simulink model "Test1_3"  (R2021a)
(part 1 of 2)
settings: Solver=FixedStepAuto  StartTime=0  StopTime=0.2  FixedStep=0.2  RelTol=1e-3
libraries: spsDistributedParametersLineLib x74, spsThreePhaseSeriesRLCLoadLib x25, spsThreePhaseVIMeasurementLib x5, spsGroundLib x1, spsThreePhaseSourceLib x1, spsSeriesRLCBranchLib x1, spspowerguiLib x1
settings Model: Creator=Admin  LastModifiedBy=Admin

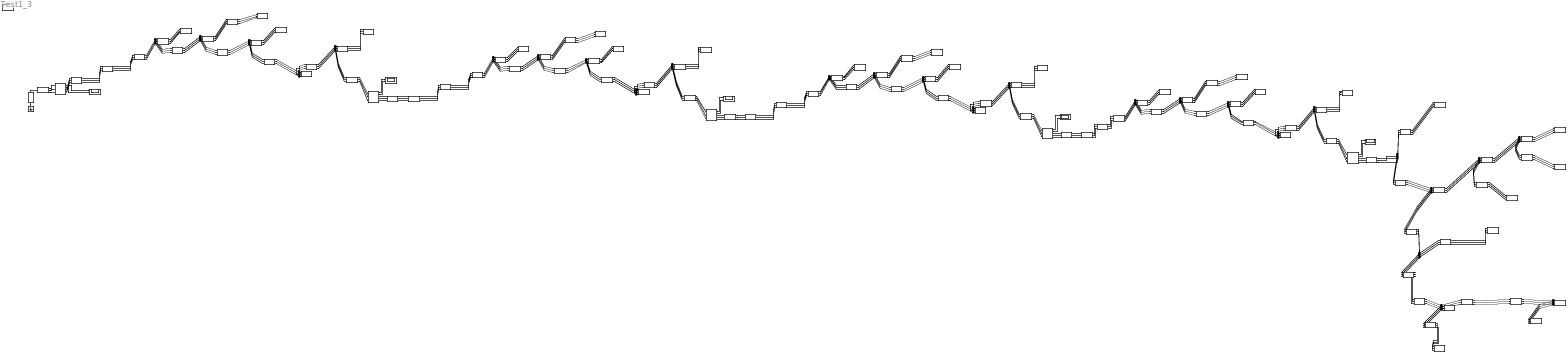
== system Test1_3 ==
  Ground : spsGroundLib/Ground  LConnTagsString=a
  Line 1 : spsDistributedParametersLineLib/Distributed Parameters Line  Phases=3  Length=0.24  Frequency=50  Resistance=[0.646656091154803 0.0486237908083191 0.0486712220507153;0.0486237908083191 0.646561225344642 0.0486237934466192;0.0486712220507153 0.0486237934466192 0.646656091154803]  Inductance=[0.00282448912315926 0.00133270803418135 0.00132951476746136;0.00133270803418135 0.00282479813276775 0.00133799988507366;0.00132951476746136 0.00133799988507366 0.00282448912315926]  Capacitance=[7.89543174552926e-09 -1.85986777702161e-09 -1.7901190036642e-09;-1.85986777702161e-09 7.82540023894543e-09 -1.8957321828871e-09;-1.7901190036642e-09 -1.8957321828871e-09 7.91264394645417e-09]  x1=[222.015092797367 9898.99389241635 9898.51429142449;314.159265358979 314.159265358979 314.159265358979;-3.07254403430719 -0.183299396266418 -1.75413682242909]  x2=[222.020723483214 9898.49942617451 9898.02069734636;314.159265358979 314.159265358979 314.159265358979;-3.07254410726608 -0.183335294452607 -1.75417253731169]  x3=[0.199348875998997 21.8526585587068 22.0454388073924;314.159265358979 314.159265358979 314.159265358979;-3.13045863300509 -0.176900643269076 -1.74803218325065]  x4=[0.189523343990307 28.5168236303326 28.7082767154191;314.159265358979 314.159265358979 314.159265358979;-3.01199407510197 -0.188487989154 -1.75911017054267]  x5=1.14995345102668e-06  V1=ones(3,3)  V2=ones(3,3)  I1=ones(3,3)  I2=ones(3,3)  nHarmo=1  Measurements=None  Decoupling=off  VsMag0=0  VrMag0=0  VsAngle0=0  VrAngle0=0  IsMag0=0  IrMag0=0  IsAngle0=0  IrAngle0=0
      settings: SourceProductBaseCode=PS
  Line 10 : spsDistributedParametersLineLib/Distributed Parameters Line  Phases=3  Length=0.17001  Frequency=50  Resistance=[0.646656091154803 0.0486237908083191 0.0486712220507153;0.0486237908083191 0.646561225344642 0.0486237934466192;0.0486712220507153 0.0486237934466192 0.646656091154803]  Inductance=[0.00282448912315926 0.00133270803418135 0.00132951476746136;0.00133270803418135 0.00282479813276775 0.00133799988507366;0.00132951476746136 0.00133799988507366 0.00282448912315926]  Capacitance=[7.89543174552926e-09 -1.85986777702161e-09 -1.7901190036642e-09;-1.85986777702161e-09 7.82540023894543e-09 -1.8957321828871e-09;-1.7901190036642e-09 -1.8957321828871e-09 7.91264394645417e-09]  x1=[221.972317308412 9904.72208898904 9904.23123830907;314.159265358979 314.159265358979 314.159265358979;-3.07236720751226 -0.182923549459791 -1.75376288206444]  x2=[221.972231728308 9904.60473873258 9904.1140740022;314.159265358979 314.159265358979 314.159265358979;-3.07237120414623 -0.182927320155413 -1.75376660852685]  x3=[0.191402295206027 24.3117265787812 24.5037810965484;314.159265358979 314.159265358979 314.159265358979;-3.07696679484423 -0.169300487327628 -1.74025339126651]  x4=[0.196725593404522 26.095480950671 26.2879206642852;314.159265358979 314.159265358979 314.159265358979;-3.06814848425652 -0.195815367857081 -1.76655565060886]  x5=8.14598275871021e-07  V1=ones(3,3)  V2=ones(3,3)  I1=ones(3,3)  I2=ones(3,3)  nHarmo=1  Measurements=None  Decoupling=off  VsMag0=0  VrMag0=0  VsAngle0=0  VrAngle0=0  IsMag0=0  IrMag0=0  IsAngle0=0  IrAngle0=0
      settings: SourceProductBaseCode=PS
  Line 11 : spsDistributedParametersLineLib/Distributed Parameters Line  Phases=3  Length=0.27998  Frequency=50  Resistance=[0.646656091154803 0.0486237908083191 0.0486712220507153;0.0486237908083191 0.646561225344642 0.0486237934466192;0.0486712220507153 0.0486237934466192 0.646656091154803]  Inductance=[0.00282448912315926 0.00133270803418135 0.00132951476746136;0.00133270803418135 0.00282479813276775 0.00133799988507366;0.00132951476746136 0.00133799988507366 0.00282448912315926]  Capacitance=[7.89543174552926e-09 -1.85986777702161e-09 -1.7901190036642e-09;-1.85986777702161e-09 7.82540023894543e-09 -1.8957321828871e-09;-1.7901190036642e-09 -1.8957321828871e-09 7.91264394645417e-09]  x1=[221.964400678937 9906.160798162 9905.66713429306;314.159265358979 314.159265358979 314.159265358979;-3.07250282075598 -0.182996515026566 -1.75383646753957]  x2=[221.972317308412 9904.72208898904 9904.23123830907;314.159265358979 314.159265358979 314.159265358979;-3.07253274376391 -0.183055057139632 -1.75389451493028]  x3=[0.189343973964793 18.3203804193673 18.510412001508;314.159265358979 314.159265358979 314.159265358979;3.11070886720037 -0.071966798330211 -1.64431562110163]  x4=[0.200581894562315 32.2574047158268 32.4491284475579;314.159265358979 314.159265358979 314.159265358979;-2.97858619624838 -0.246275175394318 -1.8165359331067]  x5=1.34151653007687e-06  V1=ones(3,3)  V2=ones(3,3)  I1=ones(3,3)  I2=ones(3,3)  nHarmo=1  Measurements=None  Decoupling=off  VsMag0=0  VrMag0=0  VsAngle0=0  VrAngle0=0  IsMag0=0  IrMag0=0  IsAngle0=0  IrAngle0=0
      settings: SourceProductBaseCode=PS
  Line 12 : spsDistributedParametersLineLib/Distributed Parameters Line  Phases=3  Length=0.01  Frequency=50  Resistance=[0.646656091154803 0.0486237908083191 0.0486712220507153;0.0486237908083191 0.646561225344642 0.0486237934466192;0.0486712220507153 0.0486237934466192 0.646656091154803]  Inductance=[0.00282448912315926 0.00133270803418135 0.00132951476746136;0.00133270803418135 0.00282479813276775 0.00133799988507366;0.00132951476746136 0.00133799988507366 0.00282448912315926]  Capacitance=[7.89543174552926e-09 -1.85986777702161e-09 -1.7901190036642e-09;-1.85986777702161e-09 7.82540023894543e-09 -1.8957321828871e-09;-1.7901190036642e-09 -1.8957321828871e-09 7.91264394645417e-09]  x1=[221.964117196425 9906.21216439256 9905.71839999673;314.159265358979 314.159265358979 314.159265358979;-3.0720953535524 -0.182671566045166 -1.75351122886673]  x2=[221.964400678937 9906.160798162 9905.66713429306;314.159265358979 314.159265358979 314.159265358979;-3.0720964237639 -0.182673659307702 -1.75351330448492]  x3=[0.189369051494013 18.3268185948226 18.5169580964303;314.159265358979 314.159265358979 314.159265358979;3.11110535727251 -0.0716738702183169 -1.64402223817255]  x4=[0.200609281456702 32.2696425742855 32.4615173065927;314.159265358979 314.159265358979 314.159265358979;-2.97774579617266 -0.245633417397122 -1.81589354797315]  x5=4.79147271261115e-08  V1=ones(3,3)  V2=ones(3,3)  I1=ones(3,3)  I2=ones(3,3)  nHarmo=1  Measurements=None  Decoupling=off  VsMag0=0  VrMag0=0  VsAngle0=0  VrAngle0=0  IsMag0=0  IrMag0=0  IsAngle0=0  IrAngle0=0
      settings: SourceProductBaseCode=PS
  Line 13 : spsDistributedParametersLineLib/Distributed Parameters Line  Phases=3  Length=0.04  Frequency=50  Resistance=[0.646656091154803 0.0486237908083191 0.0486712220507153;0.0486237908083191 0.646561225344642 0.0486237934466192;0.0486712220507153 0.0486237934466192 0.646656091154803]  Inductance=[0.00282448912315926 0.00133270803418135 0.00132951476746136;0.00133270803418135 0.00282479813276775 0.00133799988507366;0.00132951476746136 0.00133799988507366 0.00282448912315926]  Capacitance=[7.89543174552926e-09 -1.85986777702161e-09 -1.7901190036642e-09;-1.85986777702161e-09 7.82540023894543e-09 -1.8957321828871e-09;-1.7901190036642e-09 -1.8957321828871e-09 7.91264394645417e-09]  x1=[221.962982765951 9906.41761558248 9905.92344904545;314.159265358979 314.159265358979 314.159265358979;-3.07213623026815 -0.182699066907734 -1.75353883444]  x2=[221.964117196425 9906.21216439257 9905.71839999674;314.159265358979 314.159265358979 314.159265358979;-3.07214051211882 -0.182707441560263 -1.75354713853278]  x3=[0.189366364091302 18.3265238939544 18.5166548882844;314.159265358979 314.159265358979 314.159265358979;3.11100214349639 -0.071765112869428 -1.64411349403723]  x4=[0.200606435854495 32.2687271891192 32.4605884092911;314.159265358979 314.159265358979 314.159265358979;-2.97777486414768 -0.245658643022115 -1.81591879618078]  x5=1.91658908504446e-07  V1=ones(3,3)  V2=ones(3,3)  I1=ones(3,3)  I2=ones(3,3)  nHarmo=1  Measurements=None  Decoupling=off  VsMag0=0  VrMag0=0  VsAngle0=0  VrAngle0=0  IsMag0=0  IrMag0=0  IsAngle0=0  IrAngle0=0
      settings: SourceProductBaseCode=PS
  Line 14 : spsDistributedParametersLineLib/Distributed Parameters Line  Phases=3  Length=0.24  Frequency=50  Resistance=[0.646656091154803 0.0486237908083191 0.0486712220507153;0.0486237908083191 0.646561225344642 0.0486237934466192;0.0486712220507153 0.0486237934466192 0.646656091154803]  Inductance=[0.00282448912315926 0.00133270803418135 0.00132951476746136;0.00133270803418135 0.00282479813276775 0.00133799988507366;0.00132951476746136 0.00133799988507366 0.00282448912315926]  Capacitance=[7.89543174552926e-09 -1.85986777702161e-09 -1.7901190036642e-09;-1.85986777702161e-09 7.82540023894543e-09 -1.8957321828871e-09;-1.7901190036642e-09 -1.8957321828871e-09 7.91264394645417e-09]  x1=[221.973522275872 9925.87360304901 9925.32102641094;314.159265358979 314.159265358979 314.159265358979;-3.0717657082313 -0.182168328973665 -1.75301176636206]  x2=[221.977087028903 9923.47138515495 9922.92903593915;314.159265358979 314.159265358979 314.159265358979;-3.07183596694289 -0.182262149538667 -1.7531047608717]  x3=[0.166701605313396 12.4551511660944 12.6489512436628;314.159265358979 314.159265358979 314.159265358979;3.08491891689076 0.154861392301933 -1.42392082854132]  x4=[0.223729457265582 38.9654485817741 39.1305023133519;314.159265358979 314.159265358979 314.159265358979;-2.97799775422241 -0.288316615314577 -1.8579203605478]  x5=1.14995345102668e-06  V1=ones(3,3)  V2=ones(3,3)  I1=ones(3,3)  I2=ones(3,3)  nHarmo=1  Measurements=None  Decoupling=off  VsMag0=0  VrMag0=0  VsAngle0=0  VrAngle0=0  IsMag0=0  IrMag0=0  IsAngle0=0  IrAngle0=0
      settings: SourceProductBaseCode=PS
  Line 15 : spsDistributedParametersLineLib/Distributed Parameters Line  Phases=3  Length=0.17  Frequency=50  Resistance=[0.646656091154803 0.0486237908083191 0.0486712220507153;0.0486237908083191 0.646561225344642 0.0486237934466192;0.0486712220507153 0.0486237934466192 0.646656091154803]  Inductance=[0.00282448912315926 0.00133270803418135 0.00132951476746136;0.00133270803418135 0.00282479813276775 0.00133799988507366;0.00132951476746136 0.00133799988507366 0.00282448912315926]  Capacitance=[7.89543174552926e-09 -1.85986777702161e-09 -1.7901190036642e-09;-1.85986777702161e-09 7.82540023894543e-09 -1.8957321828871e-09;-1.7901190036642e-09 -1.8957321828871e-09 7.91264394645417e-09]  x1=[221.944814686174 9946.32776513441 9945.69460604376;314.159265358979 314.159265358979 314.159265358979;-3.07104566344104 -0.181319930646415 -1.75217030363738]  x2=[221.944466798057 9946.09949773542 9945.46678149026;314.159265358979 314.159265358979 314.159265358979;-3.07105307589 -0.181324540973944 -1.75217483471912]  x3=[0.188869541515534 23.713943126835 23.9061742104411;314.159265358979 314.159265358979 314.159265358979;-3.07669220860616 -0.147173041953311 -1.71830841602994]  x4=[0.199211853754603 26.9264377171524 27.1194193511748;314.159265358979 314.159265358979 314.159265358979;-3.0659487506894 -0.211587070451044 -1.78221448870695]  x5=8.14550361143895e-07  V1=ones(3,3)  V2=ones(3,3)  I1=ones(3,3)  I2=ones(3,3)  nHarmo=1  Measurements=None  Decoupling=off  VsMag0=0  VrMag0=0  VsAngle0=0  VrAngle0=0  IsMag0=0  IrMag0=0  IsAngle0=0  IrAngle0=0
      settings: SourceProductBaseCode=PS
  Line 16 : spsDistributedParametersLineLib/Distributed Parameters Line  Phases=3  Length=0.27998  Frequency=50  Resistance=[0.646656091154803 0.0486237908083191 0.0486712220507153;0.0486237908083191 0.646561225344642 0.0486237934466192;0.0486712220507153 0.0486237934466192 0.646656091154803]  Inductance=[0.00282448912315926 0.00133270803418135 0.00132951476746136;0.00133270803418135 0.00282479813276775 0.00133799988507366;0.00132951476746136 0.00133799988507366 0.00282448912315926]  Capacitance=[7.89543174552926e-09 -1.85986777702161e-09 -1.7901190036642e-09;-1.85986777702161e-09 7.82540023894543e-09 -1.8957321828871e-09;-1.7901190036642e-09 -1.8957321828871e-09 7.91264394645417e-09]  x1=[221.939122386853 9950.29824850916 9949.65104582546;314.159265358979 314.159265358979 314.159265358979;-3.07108819087539 -0.181309560588363 -1.75216142668549]  x2=[221.944814686174 9946.32776513441 9945.69460604376;314.159265358979 314.159265358979 314.159265358979;-3.07121121474554 -0.181451450284761 -1.7523019484731]  x3=[0.153632894301808 9.09985631328812 9.23355063958161;314.159265358979 314.159265358979 314.159265358979;3.01164471861859 0.584493625789448 -1.00502772438115]  x4=[0.239442202240828 44.5100191865775 44.6743802062215;314.159265358979 314.159265358979 314.159265358979;-2.94342659054599 -0.323766194698098 -1.89335245445794]  x5=1.34151653007687e-06  V1=ones(3,3)  V2=ones(3,3)  I1=ones(3,3)  I2=ones(3,3)  nHarmo=1  Measurements=None  Decoupling=off  VsMag0=0  VrMag0=0  VsAngle0=0  VrAngle0=0  IsMag0=0  IrMag0=0  IsAngle0=0  IrAngle0=0
      settings: SourceProductBaseCode=PS
  Line 17 : spsDistributedParametersLineLib/Distributed Parameters Line  Phases=3  Length=0.01  Frequency=50  Resistance=[0.646656091154803 0.0486237908083191 0.0486712220507153;0.0486237908083191 0.646561225344642 0.0486237934466192;0.0486712220507153 0.0486237934466192 0.646656091154803]  Inductance=[0.00282448912315926 0.00133270803418135 0.00132951476746136;0.00133270803418135 0.00282479813276775 0.00133799988507366;0.00132951476746136 0.00133799988507366 0.00282448912315926]  Capacitance=[7.89543174552926e-09 -1.85986777702161e-09 -1.7901190036642e-09;-1.85986777702161e-09 7.82540023894543e-09 -1.8957321828871e-09;-1.7901190036642e-09 -1.8957321828871e-09 7.91264394645417e-09]  x1=[221.938918408942 9950.44004469309 9949.79234030743;314.159265358979 314.159265358979 314.159265358979;-3.07067739832622 -0.180981636475063 -1.75183324404407]  x2=[221.939122386853 9950.29824850916 9949.65104582545;314.159265358979 314.159265358979 314.159265358979;-3.07068179388331 -0.1809867048695 -1.75183826363084]  x3=[0.153654926726157 9.10373918144453 9.23754358970651;314.159265358979 314.159265358979 314.159265358979;3.01204871867404 0.584577230830885 -1.00493947494426]  x4=[0.239480161563136 44.5300262788079 44.6945783680464;314.159265358979 314.159265358979 314.159265358979;-2.94258448112311 -0.323134577726176 -1.89272027652599]  x5=4.79147271261115e-08  V1=ones(3,3)  V2=ones(3,3)  I1=ones(3,3)  I2=ones(3,3)  nHarmo=1  Measurements=None  Decoupling=off  VsMag0=0  VrMag0=0  VsAngle0=0  VrAngle0=0  IsMag0=0  IrMag0=0  IsAngle0=0  IrAngle0=0
      settings: SourceProductBaseCode=PS
  Line 18 : spsDistributedParametersLineLib/Distributed Parameters Line  Phases=3  Length=0.04  Frequency=50  Resistance=[0.646656091154803 0.0486237908083191 0.0486712220507153;0.0486237908083191 0.646561225344642 0.0486237934466192;0.0486712220507153 0.0486237934466192 0.646656091154803]  Inductance=[0.00282448912315926 0.00133270803418135 0.00132951476746136;0.00133270803418135 0.00282479813276775 0.00133799988507366;0.00132951476746136 0.00133799988507366 0.00282448912315926]  Capacitance=[7.89543174552926e-09 -1.85986777702161e-09 -1.7901190036642e-09;-1.85986777702161e-09 7.82540023894543e-09 -1.8957321828871e-09;-1.7901190036642e-09 -1.8957321828871e-09 7.91264394645417e-09]  x1=[221.938102037263 9951.00721775521 9950.35750648626;314.159265358979 314.159265358979 314.159265358979;-3.07070497360592 -0.180997238037415 -1.75184907495375]  x2=[221.938918408942 9950.44004469309 9949.79234030743;314.159265358979 314.159265358979 314.159265358979;-3.07072255689264 -0.18101751199016 -1.75186915371012]  x3=[0.153653451843419 9.10388021603596 9.23769760590279;314.159265358979 314.159265358979 314.159265358979;3.01194864834173 0.584398219446076 -1.00511674278829]  x4=[0.239477198969098 44.5290201004338 44.6935581340705;314.159265358979 314.159265358979 314.159265358979;-2.9426134072445 -0.323160639687177 -1.89274636652624]  x5=1.91658908504446e-07  V1=ones(3,3)  V2=ones(3,3)  I1=ones(3,3)  I2=ones(3,3)  nHarmo=1  Measurements=None  Decoupling=off  VsMag0=0  VrMag0=0  VsAngle0=0  VrAngle0=0  IsMag0=0  IrMag0=0  IsAngle0=0  IrAngle0=0
      settings: SourceProductBaseCode=PS
  Line 19 : spsDistributedParametersLineLib/Distributed Parameters Line  Phases=3  Length=0.02  Frequency=50  Resistance=[0.646656091154803 0.0486237908083191 0.0486712220507153;0.0486237908083191 0.646561225344642 0.0486237934466192;0.0486712220507153 0.0486237934466192 0.646656091154803]  Inductance=[0.00282448912315926 0.00133270803418135 0.00132951476746136;0.00133270803418135 0.00282479813276775 0.00133799988507366;0.00132951476746136 0.00133799988507366 0.00282448912315926]  Capacitance=[7.89543174552926e-09 -1.85986777702161e-09 -1.7901190036642e-09;-1.85986777702161e-09 7.82540023894543e-09 -1.8957321828871e-09;-1.7901190036642e-09 -1.8957321828871e-09 7.91264394645417e-09]  x1=[221.973522275872 9925.87360304901 9925.32102641094;314.159265358979 314.159265358979 314.159265358979;-3.07143454541088 -0.181905241862953 -1.75274842881105]  x2=[221.973516698645 9925.86853585086 9925.31596800554;314.159265358979 314.159265358979 314.159265358979;-3.07143471408227 -0.181905377807733 -1.75274856290877]  x3=[0.193101763304672 24.9432757831222 25.1357901814941;314.159265358979 314.159265358979 314.159265358979;-3.07278996594042 -0.176459776755126 -1.74734653840281]  x4=[0.195053219699961 25.5768094426152 25.7694636724105;314.159265358979 314.159265358979 314.159265358979;-3.07012280847577 -0.187239577579629 -1.75804126304697]  x5=9.5829454252223e-08  V1=ones(3,3)  V2=ones(3,3)  I1=ones(3,3)  I2=ones(3,3)  nHarmo=1  Measurements=None  Decoupling=off  VsMag0=0  VrMag0=0  VsAngle0=0  VrAngle0=0  IsMag0=0  IrMag0=0  IsAngle0=0  IrAngle0=0
      settings: SourceProductBaseCode=PS
  Line 2 : spsDistributedParametersLineLib/Distributed Parameters Line  Phases=3  Length=0.02  Frequency=50  Resistance=[0.646656091154803 0.0486237908083191 0.0486712220507153;0.0486237908083191 0.646561225344642 0.0486237934466192;0.0486712220507153 0.0486237934466192 0.646656091154803]  Inductance=[0.00282448912315926 0.00133270803418135 0.00132951476746136;0.00133270803418135 0.00282479813276775 0.00133799988507366;0.00132951476746136 0.00133799988507366 0.00282448912315926]  Capacitance=[7.89543174552926e-09 -1.85986777702161e-09 -1.7901190036642e-09;-1.85986777702161e-09 7.82540023894543e-09 -1.8957321828871e-09;-1.7901190036642e-09 -1.8957321828871e-09 7.91264394645417e-09]  x1=[222.015092797367 9898.99389241635 9898.51429142449;314.159265358979 314.159265358979 314.159265358979;-3.07221287148677 -0.183036309155706 -1.75387348487807]  x2=[222.015083980034 9898.98951139534 9898.50991976959;314.159265358979 314.159265358979 314.159265358979;-3.07221300948614 -0.183036365995476 -1.75387354026733]  x3=[0.193270328840676 24.9423814090567 25.1345622020492;314.159265358979 314.159265358979 314.159265358979;-3.0727848843541 -0.177077853265056 -1.74796182768062]  x4=[0.194957058349762 25.4410435312021 25.6333539339617;314.159265358979 314.159265358979 314.159265358979;-3.07167592078859 -0.188901712894827 -1.75969386949824]  x5=9.5829454252223e-08  V1=ones(3,3)  V2=ones(3,3)  I1=ones(3,3)  I2=ones(3,3)  nHarmo=1  Measurements=None  Decoupling=off  VsMag0=0  VrMag0=0  VsAngle0=0  VrAngle0=0  IsMag0=0  IrMag0=0  IsAngle0=0  IrAngle0=0
      settings: SourceProductBaseCode=PS
  Line 20 : spsDistributedParametersLineLib/Distributed Parameters Line  Phases=3  Length=0.5  Frequency=50  Resistance=[0.646656091154803 0.0486237908083191 0.0486712220507153;0.0486237908083191 0.646561225344642 0.0486237934466192;0.0486712220507153 0.0486237934466192 0.646656091154803]  Inductance=[0.00282448912315926 0.00133270803418135 0.00132951476746136;0.00133270803418135 0.00282479813276775 0.00133799988507366;0.00132951476746136 0.00133799988507366 0.00282448912315926]  Capacitance=[7.89543174552926e-09 -1.85986777702161e-09 -1.7901190036642e-09;-1.85986777702161e-09 7.82540023894543e-09 -1.8957321828871e-09;-1.7901190036642e-09 -1.8957321828871e-09 7.91264394645417e-09]  x1=[221.966143238206 9931.00249399023 9930.42838033784;314.159265358979 314.159265358979 314.159265358979;-3.07200630035913 -0.18228019640756 -1.75312569202443]  x2=[221.973522275872 9925.87360304901 9925.32102641094;314.159265358979 314.159265358979 314.159265358979;-3.07215708247362 -0.182479250104506 -1.7533229834678]  x3=[0.165753744342144 12.2073465655838 12.3991659443851;314.159265358979 314.159265358979 314.159265358979;3.08150867253815 0.172561744291717 -1.40667076257851]  x4=[0.224703111158428 39.2896880263848 39.4545779532355;314.159265358979 314.159265358979 314.159265358979;-2.97726041033477 -0.290956906289739 -1.86055881496365]  x5=2.39573635630557e-06  V1=ones(3,3)  V2=ones(3,3)  I1=ones(3,3)  I2=ones(3,3)  nHarmo=1  Measurements=None  Decoupling=off  VsMag0=0  VrMag0=0  VsAngle0=0  VrAngle0=0  IsMag0=0  IrMag0=0  IsAngle0=0  IrAngle0=0
      settings: SourceProductBaseCode=PS
  Line 21 : spsDistributedParametersLineLib/Distributed Parameters Line  Phases=3  Length=0.23  Frequency=50  Resistance=[0.646656091154803 0.0486237908083191 0.0486712220507153;0.0486237908083191 0.646561225344642 0.0486237934466192;0.0486712220507153 0.0486237934466192 0.646656091154803]  Inductance=[0.00282448912315926 0.00133270803418135 0.00132951476746136;0.00133270803418135 0.00282479813276775 0.00133799988507366;0.00132951476746136 0.00133799988507366 0.00282448912315926]  Capacitance=[7.89543174552926e-09 -1.85986777702161e-09 -1.7901190036642e-09;-1.85986777702161e-09 7.82540023894543e-09 -1.8957321828871e-09;-1.7901190036642e-09 -1.8957321828871e-09 7.91264394645417e-09]  x1=[221.96324404488 9933.66507322255 9933.08043230388;314.159265358979 314.159265358979 314.159265358979;-3.07152069594882 -0.18186050434394 -1.75270660467828]  x2=[221.966143238206 9931.00249399023 9930.42838033784;314.159265358979 314.159265358979 314.159265358979;-3.07159987326134 -0.181957316771686 -1.75280250503001]  x3=[0.16084877950119 11.1366000486428 11.3146518193964;314.159265358979 314.159265358979 314.159265358979;3.07230850017489 0.291927218157119 -1.29006233240892]  x4=[0.229890330410908 40.9479260067839 41.1125269894925;314.159265358979 314.159265358979 314.159265358979;-2.97453896349412 -0.306501429065538 -1.87608067054056]  x5=1.10203872390056e-06  V1=ones(3,3)  V2=ones(3,3)  I1=ones(3,3)  I2=ones(3,3)  nHarmo=1  Measurements=None  Decoupling=off  VsMag0=0  VrMag0=0  VsAngle0=0  VrAngle0=0  IsMag0=0  IrMag0=0  IsAngle0=0  IrAngle0=0
      settings: SourceProductBaseCode=PS
  Line 22 : spsDistributedParametersLineLib/Distributed Parameters Line  Phases=3  Length=1.62  Frequency=50  Resistance=[0.80718830189013 0.0486237908083191 0.0486712220507153;0.0486237908083191 0.807093436079969 0.0486237934466192;0.0486712220507153 0.0486237934466192 0.80718830189013]  Inductance=[0.00279786707424938 0.00133270803418135 0.00132951476746136;0.00133270803418135 0.00279817608385787 0.00133799988507366;0.00132951476746136 0.00133799988507366 0.00279786707424938]  Capacitance=[7.73340098830622e-09 -1.79942827973291e-09 -1.73218055098733e-09;-1.79942827973291e-09 7.66505189233746e-09 -1.83375898618858e-09;-1.73218055098733e-09 -1.83375898618858e-09 7.749673531177e-09]  x1=[276.842804304554 9933.43714392975 9932.72071446311;314.159265358979 314.159265358979 314.159265358979;-2.8507933353373 -0.187817377636483 -1.75852766155098]  x2=[276.843572236788 9933.44202226371 9932.7256369537;314.159265358979 314.159265358979 314.159265358979;-2.85079548840421 -0.187820620334832 -1.75853092461075]  x3=[0.240975139197181 25.147888211045 25.3373701646833;314.159265358979 314.159265358979 314.159265358979;-2.85326877219987 -0.189597070713926 -1.76030986164388]  x4=[0.241082940762151 25.1653262960117 25.3548102521626;314.159265358979 314.159265358979 314.159265358979;-2.85074180330326 -0.187941030948555 -1.75865044109718]  x5=7.70442045759223e-06  V1=ones(3,3)  V2=ones(3,3)  I1=ones(3,3)  I2=ones(3,3)  nHarmo=1  Measurements=None  Decoupling=off  VsMag0=0  VrMag0=0  VsAngle0=0  VrAngle0=0  IsMag0=0  IrMag0=0  IsAngle0=0  IrAngle0=0
      settings: SourceProductBaseCode=PS
  Line 23 : spsDistributedParametersLineLib/Distributed Parameters Line  Phases=3  Length=0.54002  Frequency=50  Resistance=[0.646656091154803 0.0486237908083191 0.0486712220507153;0.0486237908083191 0.646561225344642 0.0486237934466192;0.0486712220507153 0.0486237934466192 0.646656091154803]  Inductance=[0.00282448912315926 0.00133270803418135 0.00132951476746136;0.00133270803418135 0.00282479813276775 0.00133799988507366;0.00132951476746136 0.00133799988507366 0.00282448912315926]  Capacitance=[7.89543174552926e-09 -1.85986777702161e-09 -1.7901190036642e-09;-1.85986777702161e-09 7.82540023894543e-09 -1.8957321828871e-09;-1.7901190036642e-09 -1.8957321828871e-09 7.91264394645417e-09]  x1=[221.955891570022 9939.90544297151 9939.29604655778;314.159265358979 314.159265358979 314.159265358979;-3.07180030545433 -0.182002080929727 -1.75285065832739]  x2=[221.96324404488 9933.66507322255 9933.08043230388;314.159265358979 314.159265358979 314.159265358979;-3.07198736457422 -0.182231241916953 -1.75307769516721]  x3=[0.160886535970452 11.1125352154197 11.2908631303351;314.159265358979 314.159265358979 314.159265358979;3.06806998069308 0.286954783554448 -1.29502772816284]  x4=[0.229926553487546 40.9440091946058 41.1084927177628;314.159265358979 314.159265358979 314.159265358979;-2.97254232875695 -0.305520532793255 -1.87509473468183]  x5=2.58749109426427e-06  V1=ones(3,3)  V2=ones(3,3)  I1=ones(3,3)  I2=ones(3,3)  nHarmo=1  Measurements=None  Decoupling=off  VsMag0=0  VrMag0=0  VsAngle0=0  VrAngle0=0  IsMag0=0  IrMag0=0  IsAngle0=0  IrAngle0=0
      settings: SourceProductBaseCode=PS
  Line 24 : spsDistributedParametersLineLib/Distributed Parameters Line  Phases=3  Length=0.13998  Frequency=50  Resistance=[0.646656091154803 0.0486237908083191 0.0486712220507153;0.0486237908083191 0.646561225344642 0.0486237934466192;0.0486712220507153 0.0486237934466192 0.646656091154803]  Inductance=[0.00282448912315926 0.00133270803418135 0.00132951476746136;0.00133270803418135 0.00282479813276775 0.00133799988507366;0.00132951476746136 0.00133799988507366 0.00282448912315926]  Capacitance=[7.89543174552926e-09 -1.85986777702161e-09 -1.7901190036642e-09;-1.85986777702161e-09 7.82540023894543e-09 -1.8957321828871e-09;-1.7901190036642e-09 -1.8957321828871e-09 7.91264394645417e-09]  x1=[221.955891570022 9939.90544297151 9939.29604655778;314.159265358979 314.159265358979 314.159265358979;-3.07119813102396 -0.181523692894413 -1.75237181490054]  x2=[221.957047427514 9939.72404212639 9939.11487634332;314.159265358979 314.159265358979 314.159265358979;-3.07120489257164 -0.18153131633055 -1.75237936601632]  x3=[0.190648933349909 23.5174842426979 23.7097126731325;314.159265358979 314.159265358979 314.159265358979;-3.10439966841434 -0.160633988569402 -1.73166517580346]  x4=[0.197658284335246 27.0755784614361 27.2685881090386;314.159265358979 314.159265358979 314.159265358979;-3.03938801160944 -0.199831408618522 -1.77053936035565]  x5=6.70710350311308e-07  V1=ones(3,3)  V2=ones(3,3)  I1=ones(3,3)  I2=ones(3,3)  nHarmo=1  Measurements=None  Decoupling=off  VsMag0=0  VrMag0=0  VsAngle0=0  VrAngle0=0  IsMag0=0  IrMag0=0  IsAngle0=0  IrAngle0=0
      settings: SourceProductBaseCode=PS
  Line 25 : spsDistributedParametersLineLib/Distributed Parameters Line  Phases=3  Length=0.14996  Frequency=50  Resistance=[0.476003738225748 0.351747138225748 0.351747138225748;0.351747138225748 0.476003738225748 0.351747138225748;0.351747138225748 0.351747138225748 0.476003738225748]  Inductance=[0.000705954362986426 0.000459934243504405 0.000459934243504405;0.000459934243504405 0.000705954362986426 0.000459934243504405;0.000459934243504405 0.000459934243504405 0.000705954362986426]  Capacitance=[5.7561313269996e-07 -1.37543883484145e-07 -1.37543912800485e-07;-1.37543883484145e-07 5.75613027339387e-07 -1.37543875208088e-07;-1.37543912800485e-07 -1.37543875208088e-07 5.75613005057695e-07]  x1=[316.03875705988 9941.21968344506 9941.46708285033;314.159265358979 314.159265358979 314.159265358979;-2.73362457165693 -0.100309086236888 -1.67109521860155]  x2=[316.038928427934 9941.1788466978 9941.42624508646;314.159265358979 314.159265358979 314.159265358979;-2.73362582380905 -0.100309919758929 -1.67109605212354]  x3=[4.28905149450592 533.056922207438 533.070146663091;314.159265358979 314.159265358979 314.159265358979;-2.73466657227107 -0.0993804469855747 -1.67016657917987]  x4=[4.28905146978253 536.612620221595 536.62593316888;314.159265358979 314.159265358979 314.159265358979;-2.73362581291863 -0.101854518161986 -1.67264065064728]  x5=3.31476347058327e-06  V1=ones(3,3)  V2=ones(3,3)  I1=ones(3,3)  I2=ones(3,3)  nHarmo=1  Measurements=None  Decoupling=off  VsMag0=0  VrMag0=0  VsAngle0=0  VrAngle0=0  IsMag0=0  IrMag0=0  IsAngle0=0  IrAngle0=0
      settings: SourceProductBaseCode=PS
  Line 26 : spsDistributedParametersLineLib/Distributed Parameters Line  Phases=3  Length=0.50001  Frequency=50  Resistance=[0.646656091154803 0.0486237908083191 0.0486712220507153;0.0486237908083191 0.646561225344642 0.0486237934466192;0.0486712220507153 0.0486237934466192 0.646656091154803]  Inductance=[0.00282448912315926 0.00133270803418135 0.00132951476746136;0.00133270803418135 0.00282479813276775 0.00133799988507366;0.00132951476746136 0.00133799988507366 0.00282448912315926]  Capacitance=[7.89543174552926e-09 -1.85986777702161e-09 -1.7901190036642e-09;-1.85986777702161e-09 7.82540023894543e-09 -1.8957321828871e-09;-1.7901190036642e-09 -1.8957321828871e-09 7.91264394645417e-09]  x1=[221.944814686174 9946.32776513441 9945.69460604376;314.159265358979 314.159265358979 314.159265358979;-3.07154242272453 -0.181714573270988 -1.75256532193378]  x2=[221.955891570022 9939.90544297151 9939.29604655778;314.159265358979 314.159265358979 314.159265358979;-3.07174007897958 -0.181954234951093 -1.75280276680277]  x3=[0.15847816303357 9.83540787761065 9.99654340404511;314.159265358979 314.159265358979 314.159265358979;3.02475647144759 0.412031916459846 -1.17353164526378]  x4=[0.234140346209793 42.7854022124726 42.9499834453038;314.159265358979 314.159265358979 314.159265358979;-2.94624307784243 -0.311180758267396 -1.88077582922916]  x5=2.3957842710327e-06  V1=ones(3,3)  V2=ones(3,3)  I1=ones(3,3)  I2=ones(3,3)  nHarmo=1  Measurements=None  Decoupling=off  VsMag0=0  VrMag0=0  VsAngle0=0  VrAngle0=0  IsMag0=0  IrMag0=0  IsAngle0=0  IrAngle0=0
      settings: SourceProductBaseCode=PS
  Line 27 : spsDistributedParametersLineLib/Distributed Parameters Line  Phases=3  Length=0.24001  Frequency=50  Resistance=[0.646656091154803 0.0486237908083191 0.0486712220507153;0.0486237908083191 0.646561225344642 0.0486237934466192;0.0486712220507153 0.0486237934466192 0.646656091154803]  Inductance=[0.00282448912315926 0.00133270803418135 0.00132951476746136;0.00133270803418135 0.00282479813276775 0.00133799988507366;0.00132951476746136 0.00133799988507366 0.00282448912315926]  Capacitance=[7.89543174552926e-09 -1.85986777702161e-09 -1.7901190036642e-09;-1.85986777702161e-09 7.82540023894543e-09 -1.8957321828871e-09;-1.7901190036642e-09 -1.8957321828871e-09 7.91264394645417e-09]  x1=[221.965094555543 9907.65140067803 9907.15307831145;314.159265358979 314.159265358979 314.159265358979;-3.07239424199511 -0.182888066532842 -1.75372813688929]  x2=[221.962982765956 9906.41761558302 9905.92344904595;314.159265358979 314.159265358979 314.159265358979;-3.07243730243036 -0.182938248966865 -1.75377824418352]  x3=[0.172738303791619 18.3230976523511 18.5067719208583;314.159265358979 314.159265358979 314.159265358979;-3.09633986630374 -0.071767125703639 -1.6452126172873]  x4=[0.21544591203728 32.2653133742822 32.4599147288413;314.159265358979 314.159265358979 314.159265358979;-3.05356025183379 -0.246168233771229 -1.81577989777661]  x5=1.1500013657538e-06  V1=ones(3,3)  V2=ones(3,3)  I1=ones(3,3)  I2=ones(3,3)  nHarmo=1  Measurements=None  Decoupling=off  VsMag0=0  VrMag0=0  VsAngle0=0  VrAngle0=0  IsMag0=0  IrMag0=0  IsAngle0=0  IrAngle0=0
      settings: SourceProductBaseCode=PS
  Line 28 : spsDistributedParametersLineLib/Distributed Parameters Line  Phases=3  Length=0.17001  Frequency=50  Resistance=[0.646656091154803 0.0486237908083191 0.0486712220507153;0.0486237908083191 0.646561225344642 0.0486237934466192;0.0486712220507153 0.0486237934466192 0.646656091154803]  Inductance=[0.00282448912315926 0.00133270803418135 0.00132951476746136;0.00133270803418135 0.00282479813276775 0.00133799988507366;0.00132951476746136 0.00133799988507366 0.00282448912315926]  Capacitance=[7.89543174552926e-09 -1.85986777702161e-09 -1.7901190036642e-09;-1.85986777702161e-09 7.82540023894543e-09 -1.8957321828871e-09;-1.7901190036642e-09 -1.8957321828871e-09 7.91264394645417e-09]  x1=[221.976691583538 9920.16930118526 9919.63509747318;314.159265358979 314.159265358979 314.159265358979;-3.07184767238349 -0.182306803799226 -1.75314862798456]  x2=[221.976594914327 9919.95535429012 9919.42146073512;314.159265358979 314.159265358979 314.159265358979;-3.07185506886873 -0.182314632447779 -1.7531563735534]  x3=[0.189224732851153 23.5750918526862 23.767152654066;314.159265358979 314.159265358979 314.159265358979;-3.08128609101912 -0.159071734056685 -1.7301134366512]  x4=[0.198923012764651 26.9180985236412 27.1108456616873;314.159265358979 314.159265358979 314.159265358979;-3.0631263242169 -0.202853873139365 -1.77354060562633]  x5=8.14598275871021e-07  V1=ones(3,3)  V2=ones(3,3)  I1=ones(3,3)  I2=ones(3,3)  nHarmo=1  Measurements=None  Decoupling=off  VsMag0=0  VrMag0=0  VsAngle0=0  VrAngle0=0  IsMag0=0  IrMag0=0  IsAngle0=0  IrAngle0=0
      settings: SourceProductBaseCode=PS
  Line 29 : spsDistributedParametersLineLib/Distributed Parameters Line  Phases=3  Length=0.27999  Frequency=50  Resistance=[0.646656091154803 0.0486237908083191 0.0486712220507153;0.0486237908083191 0.646561225344642 0.0486237934466192;0.0486712220507153 0.0486237934466192 0.646656091154803]  Inductance=[0.00282448912315926 0.00133270803418135 0.00132951476746136;0.00133270803418135 0.00282479813276775 0.00133799988507366;0.00132951476746136 0.00133799988507366 0.00282448912315926]  Capacitance=[7.89543174552926e-09 -1.85986777702161e-09 -1.7901190036642e-09;-1.85986777702161e-09 7.82540023894543e-09 -1.8957321828871e-09;-1.7901190036642e-09 -1.8957321828871e-09 7.91264394645417e-09]  x1=[221.977030436277 9922.97114305057 9922.43002833924;314.159265358979 314.159265358979 314.159265358979;-3.07191390708362 -0.182329426681661 -1.7531719764929]  x2=[221.976691583538 9920.16930118526 9919.63509747318;314.159265358979 314.159265358979 314.159265358979;-3.07201322368799 -0.182438323437571 -1.75328027282029]  x3=[0.156070100923628 12.4721553337531 12.6386914875394;314.159265358979 314.159265358979 314.159265358979;3.10808944178423 0.155849197200455 -1.42209641708897]  x4=[0.233418541306339 38.9384266609932 39.1324597301999;314.159265358979 314.159265358979 314.159265358979;-3.00342538912831 -0.28908700876416 -1.85864104412992]  x5=1.341564444804e-06  V1=ones(3,3)  V2=ones(3,3)  I1=ones(3,3)  I2=ones(3,3)  nHarmo=1  Measurements=None  Decoupling=off  VsMag0=0  VrMag0=0  VsAngle0=0  VrAngle0=0  IsMag0=0  IrMag0=0  IsAngle0=0  IrAngle0=0
      settings: SourceProductBaseCode=PS
  Line 3 : spsDistributedParametersLineLib/Distributed Parameters Line  Phases=3  Length=0.5  Frequency=50  Resistance=[0.646656091154803 0.0486237908083191 0.0486712220507153;0.0486237908083191 0.646561225344642 0.0486237934466192;0.0486712220507153 0.0486237934466192 0.646656091154803]  Inductance=[0.00282448912315926 0.00133270803418135 0.00132951476746136;0.00133270803418135 0.00282479813276775 0.00133799988507366;0.00132951476746136 0.00133799988507366 0.00282448912315926]  Capacitance=[7.89543174552926e-09 -1.85986777702161e-09 -1.7901190036642e-09;-1.85986777702161e-09 7.82540023894543e-09 -1.8957321828871e-09;-1.7901190036642e-09 -1.8957321828871e-09 7.91264394645417e-09]  x1=[222.003487056207 9900.13090845761 9899.64925086188;314.159265358979 314.159265358979 314.159265358979;-3.07293162070548 -0.183533775337669 -1.7543719126072]  x2=[222.015092797367 9898.99389241635 9898.51429142449;314.159265358979 314.159265358979 314.159265358979;-3.07293540854951 -0.183610317397259 -1.75444803953483]  x3=[0.198486971098523 21.6007974390386 21.7933753911361;314.159265358979 314.159265358979 314.159265358979;-3.13238821307855 -0.170868152695551 -1.74206655619919]  x4=[0.190346935512589 28.7602619543215 28.9516353978751;314.159265358979 314.159265358979 314.159265358979;-3.01170194618676 -0.193636962030856 -1.76422599165061]  x5=2.39573635630557e-06  V1=ones(3,3)  V2=ones(3,3)  I1=ones(3,3)  I2=ones(3,3)  nHarmo=1  Measurements=None  Decoupling=off  VsMag0=0  VrMag0=0  VsAngle0=0  VrAngle0=0  IsMag0=0  IrMag0=0  IsAngle0=0  IrAngle0=0
      settings: SourceProductBaseCode=PS
  Line 30 : spsDistributedParametersLineLib/Distributed Parameters Line  Phases=3  Length=0.01  Frequency=50  Resistance=[0.646656091154803 0.0486237908083191 0.0486712220507153;0.0486237908083191 0.646561225344642 0.0486237934466192;0.0486712220507153 0.0486237934466192 0.646656091154803]  Inductance=[0.00282448912315926 0.00133270803418135 0.00132951476746136;0.00133270803418135 0.00282479813276775 0.00133799988507366;0.00132951476746136 0.00133799988507366 0.00282448912315926]  Capacitance=[7.89543174552926e-09 -1.85986777702161e-09 -1.7901190036642e-09;-1.85986777702161e-09 7.82540023894543e-09 -1.8957321828871e-09;-1.7901190036642e-09 -1.8957321828871e-09 7.91264394645417e-09]  x1=[221.977041849809 9923.07119400891 9922.52983240527;314.159265358979 314.159265358979 314.159265358979;-3.07150394647905 -0.182002668195001 -1.75284493207239]  x2=[221.977030436277 9922.97114305057 9922.43002833924;314.159265358979 314.159265358979 314.159265358979;-3.07150749503869 -0.182006559004293 -1.75284880146836]  x3=[0.156092476561892 12.4773361771999 12.6439717344742;314.159265358979 314.159265358979 314.159265358979;3.10848724043416 0.156080941548286 -1.42186291577335]  x4=[0.233454719970261 38.9549012918942 39.1491179656434;314.159265358979 314.159265358979 314.159265358979;-3.00258962615654 -0.288451594693316 -1.85800495883342]  x5=4.79147271261115e-08  V1=ones(3,3)  V2=ones(3,3)  I1=ones(3,3)  I2=ones(3,3)  nHarmo=1  Measurements=None  Decoupling=off  VsMag0=0  VrMag0=0  VsAngle0=0  VrAngle0=0  IsMag0=0  IrMag0=0  IsAngle0=0  IrAngle0=0
      settings: SourceProductBaseCode=PS
  Line 31 : spsDistributedParametersLineLib/Distributed Parameters Line  Phases=3  Length=0.04  Frequency=50  Resistance=[0.646656091154803 0.0486237908083191 0.0486712220507153;0.0486237908083191 0.646561225344642 0.0486237934466192;0.0486712220507153 0.0486237934466192 0.646656091154803]  Inductance=[0.00282448912315926 0.00133270803418135 0.00132951476746136;0.00133270803418135 0.00282479813276775 0.00133799988507366;0.00132951476746136 0.00133799988507366 0.00282448912315926]  Capacitance=[7.89543174552926e-09 -1.85986777702161e-09 -1.7901190036642e-09;-1.85986777702161e-09 7.82540023894543e-09 -1.8957321828871e-09;-1.7901190036642e-09 -1.8957321828871e-09 7.91264394645417e-09]  x1=[221.9770870289 9923.47138515393 9922.92903593815;314.159265358979 314.159265358979 314.159265358979;-3.07153490983345 -0.182022979438057 -1.75286536309809]  x2=[221.977041849809 9923.07119400891 9922.52983240527;314.159265358979 314.159265358979 314.159265358979;-3.07154910504548 -0.182038543710098 -1.75288084173844]  x3=[0.156090976552462 12.4774700823202 12.644104602196;314.159265358979 314.159265358979 314.159265358979;3.10838457254441 0.155964041754935 -1.4219792828348]  x4=[0.233451762583562 38.9539363826219 39.1481390978754;314.159265358979 314.159265358979 314.159265358979;-3.0026190803904 -0.288477345465123 -1.85803072860756]  x5=1.91658908504446e-07  V1=ones(3,3)  V2=ones(3,3)  I1=ones(3,3)  I2=ones(3,3)  nHarmo=1  Measurements=None  Decoupling=off  VsMag0=0  VrMag0=0  VsAngle0=0  VrAngle0=0  IsMag0=0  IrMag0=0  IsAngle0=0  IrAngle0=0
      settings: SourceProductBaseCode=PS
  Line 32 : spsDistributedParametersLineLib/Distributed Parameters Line  Phases=3  Length=0.02  Frequency=50  Resistance=[0.646656091154803 0.0486237908083191 0.0486712220507153;0.0486237908083191 0.646561225344642 0.0486237934466192;0.0486712220507153 0.0486237934466192 0.646656091154803]  Inductance=[0.00282448912315926 0.00133270803418135 0.00132951476746136;0.00133270803418135 0.00282479813276775 0.00133799988507366;0.00132951476746136 0.00133799988507366 0.00282448912315926]  Capacitance=[7.89543174552926e-09 -1.85986777702161e-09 -1.7901190036642e-09;-1.85986777702161e-09 7.82540023894543e-09 -1.8957321828871e-09;-1.7901190036642e-09 -1.8957321828871e-09 7.91264394645417e-09]  x1=[221.965094555543 9907.65140067803 9907.15307831145;314.159265358979 314.159265358979 314.159265358979;-3.07206306412183 -0.182624967463625 -1.75346478736839]  x2=[221.965094059664 9907.64859258913 9907.15027393888;314.159265358979 314.159265358979 314.159265358979;-3.07206316272835 -0.182625082105148 -1.75346490088924]  x3=[0.19352887365093 25.022055751655 25.2143874461698;314.159265358979 314.159265358979 314.159265358979;-3.07320974316644 -0.180423829794984 -1.7512817790984]  x4=[0.194611278587475 25.4046782537547 25.5970861287501;314.159265358979 314.159265358979 314.159265358979;-3.07095288405867 -0.184816804376343 -1.75563903138778]  x5=9.5829454252223e-08  V1=ones(3,3)  V2=ones(3,3)  I1=ones(3,3)  I2=ones(3,3)  nHarmo=1  Measurements=None  Decoupling=off  VsMag0=0  VrMag0=0  VsAngle0=0  VrAngle0=0  IsMag0=0  IrMag0=0  IsAngle0=0  IrAngle0=0
      settings: SourceProductBaseCode=PS
  Line 33 : spsDistributedParametersLineLib/Distributed Parameters Line  Phases=3  Length=0.5  Frequency=50  Resistance=[0.646656091154803 0.0486237908083191 0.0486712220507153;0.0486237908083191 0.646561225344642 0.0486237934466192;0.0486712220507153 0.0486237934466192 0.646656091154803]  Inductance=[0.00282448912315926 0.00133270803418135 0.00132951476746136;0.00133270803418135 0.00282479813276775 0.00133799988507366;0.00132951476746136 0.00133799988507366 0.00282448912315926]  Capacitance=[7.89543174552926e-09 -1.85986777702161e-09 -1.7901190036642e-09;-1.85986777702161e-09 7.82540023894543e-09 -1.8957321828871e-09;-1.7901190036642e-09 -1.8957321828871e-09 7.91264394645417e-09]  x1=[221.969412143515 9910.2892726374 9909.78219447756;314.159265358979 314.159265358979 314.159265358979;-3.07269324751044 -0.183091263263908 -1.75393181100588]  x2=[221.965094555543 9907.65140067803 9907.15307831145;314.159265358979 314.159265358979 314.159265358979;-3.07278560118458 -0.183198975705178 -1.75403934202515]  x3=[0.172187118462172 18.138445849667 18.321827137115;314.159265358979 314.159265358979 314.159265358979;-3.09883921276452 -0.0685950364482177 -1.64210916968949]  x4=[0.21596827201466 32.4534022345412 32.6478813809388;314.159265358979 314.159265358979 314.159265358979;-3.05260782598531 -0.247536988936697 -1.81714676608442]  x5=2.39573635630557e-06  V1=ones(3,3)  V2=ones(3,3)  I1=ones(3,3)  I2=ones(3,3)  nHarmo=1  Measurements=None  Decoupling=off  VsMag0=0  VrMag0=0  VsAngle0=0  VrAngle0=0  IsMag0=0  IrMag0=0  IsAngle0=0  IrAngle0=0
      settings: SourceProductBaseCode=PS
  Line 34 : spsDistributedParametersLineLib/Distributed Parameters Line  Phases=3  Length=0.23  Frequency=50  Resistance=[0.646656091154803 0.0486237908083191 0.0486712220507153;0.0486237908083191 0.646561225344642 0.0486237934466192;0.0486712220507153 0.0486237934466192 0.646656091154803]  Inductance=[0.00282448912315926 0.00133270803418135 0.00132951476746136;0.00133270803418135 0.00282479813276775 0.00133799988507366;0.00132951476746136 0.00133799988507366 0.00282448912315926]  Capacitance=[7.89543174552926e-09 -1.85986777702161e-09 -1.7901190036642e-09;-1.85986777702161e-09 7.82540023894543e-09 -1.8957321828871e-09;-1.7901190036642e-09 -1.8957321828871e-09 7.91264394645417e-09]  x1=[221.971616485942 9911.93516644563 9911.42341005021;314.159265358979 314.159265358979 314.159265358979;-3.07222940497256 -0.182703642400711 -1.75354413180426]  x2=[221.969412143515 9910.2892726374 9909.78219447756;314.159265358979 314.159265358979 314.159265358979;-3.07228682041265 -0.182768383628034 -1.75360862401145]  x3=[0.165045761592737 15.8270953958894 16.0061019106391;314.159265358979 314.159265358979 314.159265358979;-3.11490709983858 0.00331115215524256 -1.57142132722837]  x4=[0.223322805287829 35.0014145064385 35.1957079502068;314.159265358979 314.159265358979 314.159265358979;-3.0410439003087 -0.266675863322174 -1.83625137003197]  x5=1.10203872390056e-06  V1=ones(3,3)  V2=ones(3,3)  I1=ones(3,3)  I2=ones(3,3)  nHarmo=1  Measurements=None  Decoupling=off  VsMag0=0  VrMag0=0  VsAngle0=0  VrAngle0=0  IsMag0=0  IrMag0=0  IsAngle0=0  IrAngle0=0
      settings: SourceProductBaseCode=PS
  Line 35 : spsDistributedParametersLineLib/Distributed Parameters Line  Phases=3  Length=1.62  Frequency=50  Resistance=[0.80718830189013 0.0486237908083191 0.0486712220507153;0.0486237908083191 0.807093436079969 0.0486237934466192;0.0486712220507153 0.0486237934466192 0.80718830189013]  Inductance=[0.00279786707424938 0.00133270803418135 0.00132951476746136;0.00133270803418135 0.00279817608385787 0.00133799988507366;0.00132951476746136 0.00133799988507366 0.00279786707424938]  Capacitance=[7.73340098830622e-09 -1.79942827973291e-09 -1.73218055098733e-09;-1.79942827973291e-09 7.66505189233746e-09 -1.83375898618858e-09;-1.73218055098733e-09 -1.83375898618858e-09 7.749673531177e-09]  x1=[276.725585688353 9911.70740478195 9911.06380058971;314.159265358979 314.159265358979 314.159265358979;-2.85192349579567 -0.188660565793081 -1.75936502211449]  x2=[276.726254135663 9911.69993118685 9911.05639990895;314.159265358979 314.159265358979 314.159265358979;-2.85192612114048 -0.188663573123363 -1.75936804660097]  x3=[0.240821564104113 25.0863899771267 25.2756382347359;314.159265358979 314.159265358979 314.159265358979;-2.85436401492362 -0.19020801504911 -1.76091669513618]  x4=[0.241032299003041 25.1167230703731 25.3059751962462;314.159265358979 314.159265358979 314.159265358979;-2.85190786284684 -0.1890163735874 -1.75971823804097]  x5=7.70442045759223e-06  V1=ones(3,3)  V2=ones(3,3)  I1=ones(3,3)  I2=ones(3,3)  nHarmo=1  Measurements=None  Decoupling=off  VsMag0=0  VrMag0=0  VsAngle0=0  VrAngle0=0  IsMag0=0  IrMag0=0  IsAngle0=0  IrAngle0=0
      settings: SourceProductBaseCode=PS
  Line 36 : spsDistributedParametersLineLib/Distributed Parameters Line  Phases=3  Length=0.54002  Frequency=50  Resistance=[0.646656091154803 0.0486237908083191 0.0486712220507153;0.0486237908083191 0.646561225344642 0.0486237934466192;0.0486712220507153 0.0486237934466192 0.646656091154803]  Inductance=[0.00282448912315926 0.00133270803418135 0.00132951476746136;0.00133270803418135 0.00282479813276775 0.00133799988507366;0.00132951476746136 0.00133799988507366 0.00282448912315926]  Capacitance=[7.89543174552926e-09 -1.85986777702161e-09 -1.7901190036642e-09;-1.85986777702161e-09 7.82540023894543e-09 -1.8957321828871e-09;-1.7901190036642e-09 -1.8957321828871e-09 7.91264394645417e-09]  x1=[221.976255959453 9915.79184660861 9915.26906363002;314.159265358979 314.159265358979 314.159265358979;-3.07256001901775 -0.182920424049955 -1.75376183687469]  x2=[221.971616485942 9911.93516644563 9911.42341005021;314.159265358979 314.159265358979 314.159265358979;-3.07269607359796 -0.183074379973724 -1.75391522229319]  x3=[0.165009681637327 15.8057298240534 15.9847615515989;314.159265358979 314.159265358979 314.159265358979;-3.1191178695848 -0.000149371082823487 -1.5748842968228]  x4=[0.223352030627783 35.005580933905 35.1997666389744;314.159265358979 314.159265358979 314.159265358979;-3.03899420006866 -0.265657046793187 -1.83522782969093]  x5=2.58749109426427e-06  V1=ones(3,3)  V2=ones(3,3)  I1=ones(3,3)  I2=ones(3,3)  nHarmo=1  Measurements=None  Decoupling=off  VsMag0=0  VrMag0=0  VsAngle0=0  VrAngle0=0  IsMag0=0  IrMag0=0  IsAngle0=0  IrAngle0=0
      settings: SourceProductBaseCode=PS
  Line 37 : spsDistributedParametersLineLib/Distributed Parameters Line  Phases=3  Length=0.13998  Frequency=50  Resistance=[0.646656091154803 0.0486237908083191 0.0486712220507153;0.0486237908083191 0.646561225344642 0.0486237934466192;0.0486712220507153 0.0486237934466192 0.646656091154803]  Inductance=[0.00282448912315926 0.00133270803418135 0.00132951476746136;0.00133270803418135 0.00282479813276775 0.00133799988507366;0.00132951476746136 0.00133799988507366 0.00282448912315926]  Capacitance=[7.89543174552926e-09 -1.85986777702161e-09 -1.7901190036642e-09;-1.85986777702161e-09 7.82540023894543e-09 -1.8957321828871e-09;-1.7901190036642e-09 -1.8957321828871e-09 7.91264394645417e-09]  x1=[221.976255959453 9915.79184660861 9915.26906363002;314.159265358979 314.159265358979 314.159265358979;-3.07195784458738 -0.18244203601464 -1.75328299344784]  x2=[221.977296364838 9915.56495941441 9915.04251269154;314.159265358979 314.159265358979 314.159265358979;-3.07196599577977 -0.182449927686265 -1.75329079838955]  x3=[0.189415601438106 23.1124444136863 23.3042528091546;314.159265358979 314.159265358979 314.159265358979;-3.10570151837491 -0.150549234893659 -1.72166789533243]  x4=[0.1989311915227 27.3699181209043 27.5627479342293;314.159265358979 314.159265358979 314.159265358979;-3.04004244677455 -0.209534155921971 -1.78017404125904]  x5=6.70710350311308e-07  V1=ones(3,3)  V2=ones(3,3)  I1=ones(3,3)  I2=ones(3,3)  nHarmo=1  Measurements=None  Decoupling=off  VsMag0=0  VrMag0=0  VsAngle0=0  VrAngle0=0  IsMag0=0  IrMag0=0  IsAngle0=0  IrAngle0=0
      settings: SourceProductBaseCode=PS
  Line 38 : spsDistributedParametersLineLib/Distributed Parameters Line  Phases=3  Length=0.14997  Frequency=50  Resistance=[0.476003738225748 0.351747138225748 0.351747138225748;0.351747138225748 0.476003738225748 0.351747138225748;0.351747138225748 0.351747138225748 0.476003738225748]  Inductance=[0.000705954362986426 0.000459934243504405 0.000459934243504405;0.000459934243504405 0.000705954362986426 0.000459934243504405;0.000459934243504405 0.000459934243504405 0.000705954362986426]  Capacitance=[5.7561313269996e-07 -1.37543883484145e-07 -1.37543912800485e-07;-1.37543883484145e-07 5.75613027339387e-07 -1.37543875208088e-07;-1.37543912800485e-07 -1.37543875208088e-07 5.75613005057695e-07]  x1=[315.810671683347 9917.05281799241 9917.39452677272;314.159265358979 314.159265358979 314.159265358979;-2.73502350302124 -0.101226966778527 -1.67200755922329]  x2=[315.810842951588 9917.00260678372 9917.34431383358;314.159265358979 314.159265358979 314.159265358979;-2.7350247553459 -0.10122775091135 -1.67200834335606]  x3=[4.28595556949605 531.406853063994 531.425122365906;314.159265358979 314.159265358979 314.159265358979;-2.7360655755901 -0.0998333145428434 -1.67061390677999]  x4=[4.28595554222782 535.662509603149 535.680925544425;314.159265358979 314.159265358979 314.159265358979;-2.73502474201568 -0.103232073170151 -1.67401266577165]  x5=3.31498451375949e-06  V1=ones(3,3)  V2=ones(3,3)  I1=ones(3,3)  I2=ones(3,3)  nHarmo=1  Measurements=None  Decoupling=off  VsMag0=0  VrMag0=0  VsAngle0=0  VrAngle0=0  IsMag0=0  IrMag0=0  IsAngle0=0  IrAngle0=0
      settings: SourceProductBaseCode=PS
  Line 39 : spsDistributedParametersLineLib/Distributed Parameters Line  Phases=3  Length=0.50001  Frequency=50  Resistance=[0.646656091154803 0.0486237908083191 0.0486712220507153;0.0486237908083191 0.646561225344642 0.0486237934466192;0.0486712220507153 0.0486237934466192 0.646656091154803]  Inductance=[0.00282448912315926 0.00133270803418135 0.00132951476746136;0.00133270803418135 0.00282479813276775 0.00133799988507366;0.00132951476746136 0.00133799988507366 0.00282448912315926]  Capacitance=[7.89543174552926e-09 -1.85986777702161e-09 -1.7901190036642e-09;-1.85986777702161e-09 7.82540023894543e-09 -1.8957321828871e-09;-1.7901190036642e-09 -1.8957321828871e-09 7.91264394645417e-09]  x1=[221.976691583538 9920.16930118526 9919.63509747318;314.159265358979 314.159265358979 314.159265358979;-3.07234441661413 -0.182701434465293 -1.75354363431108]  x2=[221.976255959453 9915.79184660861 9915.26906363002;314.159265358979 314.159265358979 314.159265358979;-3.072499792543 -0.18287257807132 -1.75371394535007]  x3=[0.160701921954316 13.8991703051462 14.0722788376741;314.159265358979 314.159265358979 314.159265358979;3.12229932262638 0.0790397444700069 -1.49724017774692]  x4=[0.228428189290569 37.2019239369732 37.3959541511308;314.159265358979 314.159265358979 314.159265358979;-3.01086838751989 -0.280054173259507 -1.84960967027726]  x5=2.3957842710327e-06  V1=ones(3,3)  V2=ones(3,3)  I1=ones(3,3)  I2=ones(3,3)  nHarmo=1  Measurements=None  Decoupling=off  VsMag0=0  VrMag0=0  VsAngle0=0  VrAngle0=0  IsMag0=0  IrMag0=0  IsAngle0=0  IrAngle0=0
      settings: SourceProductBaseCode=PS
  Line 4 : spsDistributedParametersLineLib/Distributed Parameters Line  Phases=3  Length=0.23  Frequency=50  Resistance=[0.646656091154803 0.0486237908083191 0.0486712220507153;0.0486237908083191 0.646561225344642 0.0486237934466192;0.0486712220507153 0.0486237934466192 0.646656091154803]  Inductance=[0.00282448912315926 0.00133270803418135 0.00132951476746136;0.00133270803418135 0.00282479813276775 0.00133799988507366;0.00132951476746136 0.00133799988507366 0.00282448912315926]  Capacitance=[7.89543174552926e-09 -1.85986777702161e-09 -1.7901190036642e-09;-1.85986777702161e-09 7.82540023894543e-09 -1.8957321828871e-09;-1.7901190036642e-09 -1.8957321828871e-09 7.91264394645417e-09]  x1=[221.998599971118 9900.83919865606 9900.35614301331;314.159265358979 314.159265358979 314.159265358979;-3.07251773275133 -0.183174889728172 -1.75401296674876]  x2=[222.003487056207 9900.13090845761 9899.64925086188;314.159265358979 314.159265358979 314.159265358979;-3.07252519360769 -0.183210895701795 -1.75404872561278]  x3=[0.195406518553412 20.76661255207 20.9587367048412;314.159265358979 314.159265358979 314.159265358979;-3.13376282237124 -0.139991024906718 -1.71149010379653]  x4=[0.193488693151401 29.6446162704774 29.8361822574686;314.159265358979 314.159265358979 314.159265358979;-3.01102027021331 -0.213685653231737 -1.7841437913132]  x5=1.10203872390056e-06  V1=ones(3,3)  V2=ones(3,3)  I1=ones(3,3)  I2=ones(3,3)  nHarmo=1  Measurements=None  Decoupling=off  VsMag0=0  VrMag0=0  VsAngle0=0  VrAngle0=0  IsMag0=0  IrMag0=0  IsAngle0=0  IrAngle0=0
      settings: SourceProductBaseCode=PS
  Line 44 : spsDistributedParametersLineLib/Distributed Parameters Line  Phases=3  Length=1.11  Frequency=50  Resistance=[0.502970710632245 0.0486237908083191 0.0486712220507153;0.0486237908083191 0.502875844822084 0.0486237934466192;0.0486712220507153 0.0486237934466192 0.502970710632245]  Inductance=[0.00286900545038753 0.00133270803418135 0.00132951476746136;0.00133270803418135 0.00286931445999602 0.00133799988507366;0.00132951476746136 0.00133799988507366 0.00286900545038753]  Capacitance=[8.11484299003193e-09 -1.94249816214699e-09 -1.86930692621136e-09;-1.94249816214699e-09 8.0425699231653e-09 -1.98049571960044e-09;-1.86930692621136e-09 -1.98049571960044e-09 8.13337738722527e-09]  x1=[177.860922565512 9894.78010878648 9894.41288926103;314.159265358979 314.159265358979 314.159265358979;2.72736794848087 -0.178423113372315 -1.7494184297498]  x2=[177.86117615637 9894.78936196175 9894.4221629306;314.159265358979 314.159265358979 314.159265358979;2.72736745626916 -0.178423991174418 -1.74941931511305]  x3=[0.155929407422012 25.1701843789931 25.3625065903367;314.159265358979 314.159265358979 314.159265358979;2.72567904597649 -0.17979114636586 -1.75078800559586]  x4=[0.155929407486935 25.1701843864938 25.3625065980017;314.159265358979 314.159265358979 314.159265358979;2.72736745631776 -0.178423991173072 -1.74941931511453]  x5=5.37516004033389e-06  V1=ones(3,3)  V2=ones(3,3)  I1=ones(3,3)  I2=ones(3,3)  nHarmo=1  Measurements=None  Decoupling=off  VsMag0=0  VrMag0=0  VsAngle0=0  VrAngle0=0  IsMag0=0  IrMag0=0  IsAngle0=0  IrAngle0=0
      settings: SourceProductBaseCode=PS
  Line 45 : spsDistributedParametersLineLib/Distributed Parameters Line  Phases=3  Length=0.03  Frequency=50  Resistance=[0.476003738225748 0.351747138225748 0.351747138225748;0.351747138225748 0.476003738225748 0.351747138225748;0.351747138225748 0.351747138225748 0.476003738225748]  Inductance=[0.000705954362986426 0.000459934243504405 0.000459934243504405;0.000459934243504405 0.000705954362986426 0.000459934243504405;0.000459934243504405 0.000459934243504405 0.000705954362986426]  Capacitance=[5.7561313269996e-07 -1.37543883484145e-07 -1.37543912800485e-07;-1.37543883484145e-07 5.75613027339387e-07 -1.37543875208088e-07;-1.37543912800485e-07 -1.37543875208088e-07 5.75613005057695e-07]  x1=[315.714309704931 9895.86183071986 9896.25661920576;314.159265358979 314.159265358979 314.159265358979;-2.73555341227259 -0.101760441778501 -1.67253661387823]  x2=[315.714314567943 9895.86198782501 9896.25677680231;314.159265358979 314.159265358979 314.159265358979;-2.73555349255435 -0.101760467276991 -1.67253663950117]  x3=[4.29068619764692 532.715760115087 532.736916983409;314.159265358979 314.159265358979 314.159265358979;-2.73580981614019 -0.101949952595808 -1.67272668138175]  x4=[4.29097700227886 532.715701196715 532.736966719545;314.159265358979 314.159265358979 314.159265358979;-2.73550545234375 -0.10169580134418 -1.67247141690019]  x5=6.63129528657629e-07  V1=ones(3,3)  V2=ones(3,3)  I1=ones(3,3)  I2=ones(3,3)  nHarmo=1  Measurements=None  Decoupling=off  VsMag0=0  VrMag0=0  VsAngle0=0  VrAngle0=0  IsMag0=0  IrMag0=0  IsAngle0=0  IrAngle0=0
      settings: SourceProductBaseCode=PS
  Line 46 : spsDistributedParametersLineLib/Distributed Parameters Line  Phases=3  Length=0.28003  Frequency=50  Resistance=[0.476003738225748 0.351747138225748 0.351747138225748;0.351747138225748 0.476003738225748 0.351747138225748;0.351747138225748 0.351747138225748 0.476003738225748]  Inductance=[0.000705954362986426 0.000459934243504405 0.000459934243504405;0.000459934243504405 0.000705954362986426 0.000459934243504405;0.000459934243504405 0.000459934243504405 0.000705954362986426]  Capacitance=[5.7561313269996e-07 -1.37543883484145e-07 -1.37543912800485e-07;-1.37543883484145e-07 5.75613027339387e-07 -1.37543875208088e-07;-1.37543912800485e-07 -1.37543875208088e-07 5.75613005057695e-07]  x1=[315.714309704931 9895.86183071986 9896.25661920576;314.159265358979 314.159265358979 314.159265358979;-2.73728968964721 -0.102800888583748 -1.67357706060304]  x2=[315.714895777082 9895.86909312946 9896.2638851355;314.159265358979 314.159265358979 314.159265358979;-2.73729427354208 -0.102802068276923 -1.67357824110636]  x3=[4.2778554512269 532.048301976577 532.06945048441;314.159265358979 314.159265358979 314.159265358979;-2.73927458990945 -0.104013827857063 -1.6747903900962]  x4=[4.27806164776347 532.048262564772 532.069483731432;314.159265358979 314.159265358979 314.159265358979;-2.73725621069995 -0.102754960161175 -1.67353074276655]  x5=6.18987206366653e-06  V1=ones(3,3)  V2=ones(3,3)  I1=ones(3,3)  I2=ones(3,3)  nHarmo=1  Measurements=None  Decoupling=off  VsMag0=0  VrMag0=0  VsAngle0=0  VrAngle0=0  IsMag0=0  IrMag0=0  IsAngle0=0  IrAngle0=0
      settings: SourceProductBaseCode=PS
  Line 47 : spsDistributedParametersLineLib/Distributed Parameters Line  Phases=3  Length=0.28004  Frequency=50  Resistance=[0.646656091154803 0.0486237908083191 0.0486712220507153;0.0486237908083191 0.646561225344642 0.0486237934466192;0.0486712220507153 0.0486237934466192 0.646656091154803]  Inductance=[0.00282448912315926 0.00133270803418135 0.00132951476746136;0.00133270803418135 0.00282479813276775 0.00133799988507366;0.00132951476746136 0.00133799988507366 0.00282448912315926]  Capacitance=[7.89543174552926e-09 -1.85986777702161e-09 -1.7901190036642e-09;-1.85986777702161e-09 7.82540023894543e-09 -1.8957321828871e-09;-1.7901190036642e-09 -1.8957321828871e-09 7.91264394645417e-09]  x1=[222.083958242892 9894.38736433658 9893.91242442329;314.159265358979 314.159265358979 314.159265358979;-3.07279824792137 -0.183651757725395 -1.75448737396932]  x2=[222.084057701505 9894.39011104819 9893.91517606631;314.159265358979 314.159265358979 314.159265358979;-3.07279843640744 -0.183652110929785 -1.75448773012808]  x3=[0.194151257647454 25.1720968480129 25.3641548883536;314.159265358979 314.159265358979 314.159265358979;-3.07406745101608 -0.184648264453853 -1.75548476162498]  x4=[0.194147649190284 25.1720972467247 25.3641545869961;314.159265358979 314.159265358979 314.159265358979;-3.07195077299903 -0.182990525860809 -1.75382558319863]  x5=1.34180401843963e-06  V1=ones(3,3)  V2=ones(3,3)  I1=ones(3,3)  I2=ones(3,3)  nHarmo=1  Measurements=None  Decoupling=off  VsMag0=0  VrMag0=0  VsAngle0=0  VrAngle0=0  IsMag0=0  IrMag0=0  IsAngle0=0  IrAngle0=0
      settings: SourceProductBaseCode=PS
  Line 48 : spsDistributedParametersLineLib/Distributed Parameters Line  Phases=3  Length=0.3  Frequency=50  Resistance=[0.80718830189013 0.0486237908083191 0.0486712220507153;0.0486237908083191 0.807093436079969 0.0486237934466192;0.0486712220507153 0.0486237934466192 0.80718830189013]  Inductance=[0.00279786707424938 0.00133270803418135 0.00132951476746136;0.00133270803418135 0.00279817608385787 0.00133799988507366;0.00132951476746136 0.00133799988507366 0.00279786707424938]  Capacitance=[7.73340098830622e-09 -1.79942827973291e-09 -1.73218055098733e-09;-1.79942827973291e-09 7.66505189233746e-09 -1.83375898618858e-09;-1.73218055098733e-09 -1.83375898618858e-09 7.749673531177e-09]  x1=[276.747990445267 9894.16239567018 9893.55538557065;314.159265358979 314.159265358979 314.159265358979;-2.85093217494216 -0.188002676657011 -1.75870070663958]  x2=[276.748018245413 9894.16300686091 9893.55599775703;314.159265358979 314.159265358979 314.159265358979;-2.85093222786298 -0.188002778155552 -1.75870080898336]  x3=[0.241133630256357 25.104912186617 25.294638472556;314.159265358979 314.159265358979 314.159265358979;-2.85138042660344 -0.188354218125235 -1.75905254549768]  x4=[0.241133630230461 25.104912186758 25.2946384726213;314.159265358979 314.159265358979 314.159265358979;-2.85093222769981 -0.188002778153787 -1.75870080898262]  x5=1.42674452918375e-06  V1=ones(3,3)  V2=ones(3,3)  I1=ones(3,3)  I2=ones(3,3)  nHarmo=1  Measurements=None  Decoupling=off  VsMag0=0  VrMag0=0  VsAngle0=0  VrAngle0=0  IsMag0=0  IrMag0=0  IsAngle0=0  IrAngle0=0
      settings: SourceProductBaseCode=PS
  Line 49 : spsDistributedParametersLineLib/Distributed Parameters Line  Phases=3  Length=0.25999  Frequency=50  Resistance=[0.646656091154803 0.0486237908083191 0.0486712220507153;0.0486237908083191 0.646561225344642 0.0486237934466192;0.0486712220507153 0.0486237934466192 0.646656091154803]  Inductance=[0.00282448912315926 0.00133270803418135 0.00132951476746136;0.00133270803418135 0.00282479813276775 0.00133799988507366;0.00132951476746136 0.00133799988507366 0.00282448912315926]  Capacitance=[7.89543174552926e-09 -1.85986777702161e-09 -1.7901190036642e-09;-1.85986777702161e-09 7.82540023894543e-09 -1.8957321828871e-09;-1.7901190036642e-09 -1.8957321828871e-09 7.91264394645417e-09]  x1=[222.084057701505 9894.39011104819 9893.91517606631;314.159265358979 314.159265358979 314.159265358979;-3.07276825543222 -0.183628134127195 -1.75446373050127]  x2=[222.084074708933 9894.39058926641 9893.91565517242;314.159265358979 314.159265358979 314.159265358979;-3.07276828845785 -0.183628195620883 -1.75446379251525]  x3=[0.194151293914889 25.1726686690661 25.3647350670155;314.159265358979 314.159265358979 314.159265358979;-3.07315963121464 -0.183939074047228 -1.75477496664214]  x4=[0.194151293931191 25.1726686691555 25.3647350670059;314.159265358979 314.159265358979 314.159265358979;-3.07276828832889 -0.183628195620049 -1.75446379251804]  x5=1.24573499055177e-06  V1=ones(3,3)  V2=ones(3,3)  I1=ones(3,3)  I2=ones(3,3)  nHarmo=1  Measurements=None  Decoupling=off  VsMag0=0  VrMag0=0  VsAngle0=0  VrAngle0=0  IsMag0=0  IrMag0=0  IsAngle0=0  IrAngle0=0
      settings: SourceProductBaseCode=PS
  Line 5 : spsDistributedParametersLineLib/Distributed Parameters Line  Phases=3  Length=1.62  Frequency=50  Resistance=[0.80718830189013 0.0486237908083191 0.0486712220507153;0.0486237908083191 0.807093436079969 0.0486237934466192;0.0486712220507153 0.0486237934466192 0.80718830189013]  Inductance=[0.00279786707424938 0.00133270803418135 0.00132951476746136;0.00133270803418135 0.00279817608385787 0.00133799988507366;0.00132951476746136 0.00133799988507366 0.00279786707424938]  Capacitance=[7.73340098830622e-09 -1.79942827973291e-09 -1.73218055098733e-09;-1.79942827973291e-09 7.66505189233746e-09 -1.83375898618858e-09;-1.73218055098733e-09 -1.83375898618858e-09 7.749673531177e-09]  x1=[276.693488713517 9900.61148371318 9899.99652141362;314.159265358979 314.159265358979 314.159265358979;-2.85247026789067 -0.18913183880338 -1.75983377083035]  x2=[276.694146299048 9900.6033407301 9899.98845418443;314.159265358979 314.159265358979 314.159265358979;-2.85247290830052 -0.189134785790625 -1.75983673487879]  x3=[0.240790851518435 25.0581191425366 25.2472267085979;314.159265358979 314.159265358979 314.159265358979;-2.85490076960363 -0.190655398852442 -1.76136173066098]  x4=[0.241007106798294 25.0887902973371 25.2779018809974;314.159265358979 314.159265358979 314.159265358979;-2.85246468668328 -0.18951145512866 -1.76021061959066]  x5=7.70442045759223e-06  V1=ones(3,3)  V2=ones(3,3)  I1=ones(3,3)  I2=ones(3,3)  nHarmo=1  Measurements=None  Decoupling=off  VsMag0=0  VrMag0=0  VsAngle0=0  VrAngle0=0  IsMag0=0  IrMag0=0  IsAngle0=0  IrAngle0=0
      settings: SourceProductBaseCode=PS
  Line 50 : spsDistributedParametersLineLib/Distributed Parameters Line  Phases=3  Length=0.02  Frequency=50  Resistance=[0.476003738225748 0.351747138225748 0.351747138225748;0.351747138225748 0.476003738225748 0.351747138225748;0.351747138225748 0.351747138225748 0.476003738225748]  Inductance=[0.000705954362986426 0.000459934243504405 0.000459934243504405;0.000459934243504405 0.000705954362986426 0.000459934243504405;0.000459934243504405 0.000459934243504405 0.000705954362986426]  Capacitance=[5.7561313269996e-07 -1.37543883484145e-07 -1.37543912800485e-07;-1.37543883484145e-07 5.75613027339387e-07 -1.37543875208088e-07;-1.37543912800485e-07 -1.37543875208088e-07 5.75613005057695e-07]  x1=[315.71421435895 9895.86563622173 9896.26042430539;314.159265358979 314.159265358979 314.159265358979;-2.73548322107899 -0.101718574555985 -1.67249474651812]  x2=[315.714309704931 9895.86183071986 9896.25661920576;314.159265358979 314.159265358979 314.159265358979;-2.73548396951073 -0.101718828899836 -1.67249500100278]  x3=[4.29110939734221 531.184408452328 531.205467811166;314.159265358979 314.159265358979 314.159265358979;-2.7378614342512 -0.101842166484431 -1.67261928774198]  x4=[4.29160733645256 534.300701759216 534.322066871781;314.159265358979 314.159265358979 314.159265358979;-2.7332449207586 -0.101678942903541 -1.67245417126919]  x5=4.42086352438419e-07  V1=ones(3,3)  V2=ones(3,3)  I1=ones(3,3)  I2=ones(3,3)  nHarmo=1  Measurements=None  Decoupling=off  VsMag0=0  VrMag0=0  VsAngle0=0  VrAngle0=0  IsMag0=0  IrMag0=0  IsAngle0=0  IrAngle0=0
      settings: SourceProductBaseCode=PS
  Line 51 : spsDistributedParametersLineLib/Distributed Parameters Line  Phases=3  Length=1.7101  Frequency=50  Resistance=[0.646656091154803 0.0486237908083191 0.0486712220507153;0.0486237908083191 0.646561225344642 0.0486237934466192;0.0486712220507153 0.0486237934466192 0.646656091154803]  Inductance=[0.00282448912315926 0.00133270803418135 0.00132951476746136;0.00133270803418135 0.00282479813276775 0.00133799988507366;0.00132951476746136 0.00133799988507366 0.00282448912315926]  Capacitance=[7.89543174552926e-09 -1.85986777702161e-09 -1.7901190036642e-09;-1.85986777702161e-09 7.82540023894543e-09 -1.8957321828871e-09;-1.7901190036642e-09 -1.8957321828871e-09 7.91264394645417e-09]  x1=[222.04528543322 9895.90413654009 9895.42890355539;314.159265358979 314.159265358979 314.159265358979;-3.07486675811975 -0.185224472439119 -1.75606241752747]  x2=[222.082935779284 9894.38391075076 9893.90896204154;314.159265358979 314.159265358979 314.159265358979;-3.07494508735392 -0.185360461748615 -1.75619770519094]  x3=[0.194096168296793 23.5786432723156 23.7697732446221;314.159265358979 314.159265358979 314.159265358979;3.14039470554569 -0.19017188630361 -1.7610241420477]  x4=[0.194756897359038 26.6876480586959 26.8794212841301;314.159265358979 314.159265358979 314.159265358979;-3.00982242327005 -0.182908630945281 -1.75373199184361]  x5=8.19389748583632e-06  V1=ones(3,3)  V2=ones(3,3)  I1=ones(3,3)  I2=ones(3,3)  nHarmo=1  Measurements=None  Decoupling=off  VsMag0=0  VrMag0=0  VsAngle0=0  VrAngle0=0  IsMag0=0  IrMag0=0  IsAngle0=0  IrAngle0=0
      settings: SourceProductBaseCode=PS
  Line 52 : spsDistributedParametersLineLib/Distributed Parameters Line  Phases=3  Length=0.02  Frequency=50  Resistance=[0.646656091154803 0.0486237908083191 0.0486712220507153;0.0486237908083191 0.646561225344642 0.0486237934466192;0.0486712220507153 0.0486237934466192 0.646656091154803]  Inductance=[0.00282448912315926 0.00133270803418135 0.00132951476746136;0.00133270803418135 0.00282479813276775 0.00133799988507366;0.00132951476746136 0.00133799988507366 0.00282448912315926]  Capacitance=[7.89543174552926e-09 -1.85986777702161e-09 -1.7901190036642e-09;-1.85986777702161e-09 7.82540023894543e-09 -1.8957321828871e-09;-1.7901190036642e-09 -1.8957321828871e-09 7.91264394645417e-09]  x1=[222.04528543322 9895.90413654009 9895.42890355539;314.159265358979 314.159265358979 314.159265358979;-3.07232267501612 -0.183203365503601 -1.75403938664127]  x2=[222.04526107562 9895.89451540526 9895.41930516079;314.159265358979 314.159265358979 314.159265358979;-3.07232296813011 -0.183203415355817 -1.75403943348818]  x3=[0.192289084732336 24.6687055733041 24.8607385684981;314.159265358979 314.159265358979 314.159265358979;-3.07281035550321 -0.168402215220081 -1.73935461558381]  x4=[0.195991068164965 25.7034037949149 25.8957289635479;314.159265358979 314.159265358979 314.159265358979;-3.07187431848977 -0.197432134669547 -1.7681607101652]  x5=9.5829454252223e-08  V1=ones(3,3)  V2=ones(3,3)  I1=ones(3,3)  I2=ones(3,3)  nHarmo=1  Measurements=None  Decoupling=off  VsMag0=0  VrMag0=0  VsAngle0=0  VrAngle0=0  IsMag0=0  IrMag0=0  IsAngle0=0  IrAngle0=0
      settings: SourceProductBaseCode=PS
  Line 53 : spsDistributedParametersLineLib/Distributed Parameters Line  Phases=3  Length=0.02  Frequency=50  Resistance=[0.646656091154803 0.0486237908083191 0.0486712220507153;0.0486237908083191 0.646561225344642 0.0486237934466192;0.0486712220507153 0.0486237934466192 0.646656091154803]  Inductance=[0.00282448912315926 0.00133270803418135 0.00132951476746136;0.00133270803418135 0.00282479813276775 0.00133799988507366;0.00132951476746136 0.00133799988507366 0.00282448912315926]  Capacitance=[7.89543174552926e-09 -1.85986777702161e-09 -1.7901190036642e-09;-1.85986777702161e-09 7.82540023894543e-09 -1.8957321828871e-09;-1.7901190036642e-09 -1.8957321828871e-09 7.91264394645417e-09]  x1=[222.044860664132 9895.93129049812 9895.45603097759;314.159265358979 314.159265358979 314.159265358979;-3.07232144856315 -0.183201693633047 -1.7540377257112]  x2=[222.04528543322 9895.90413654009 9895.42890355539;314.159265358979 314.159265358979 314.159265358979;-3.07232267501612 -0.183203365503601 -1.75403938664127]  x3=[0.192415551166085 23.1088546739065 23.3005317282342;314.159265358979 314.159265358979 314.159265358979;-3.14139609411318 -0.17248221519631 -1.74346413765317]  x4=[0.196771325491343 27.2605033132268 27.4531814031985;314.159265358979 314.159265358979 314.159265358979;-3.0048091949576 -0.192312236415455 -1.76303553918894]  x5=9.5829454252223e-08  V1=ones(3,3)  V2=ones(3,3)  I1=ones(3,3)  I2=ones(3,3)  nHarmo=1  Measurements=None  Decoupling=off  VsMag0=0  VrMag0=0  VsAngle0=0  VrAngle0=0  IsMag0=0  IrMag0=0  IsAngle0=0  IrAngle0=0
      settings: SourceProductBaseCode=PS
  Line 54 : spsDistributedParametersLineLib/Distributed Parameters Line  Phases=3  Length=1.15  Frequency=50  Resistance=[0.646656091154803 0.0486237908083191 0.0486712220507153;0.0486237908083191 0.646561225344642 0.0486237934466192;0.0486712220507153 0.0486237934466192 0.646656091154803]  Inductance=[0.00282448912315926 0.00133270803418135 0.00132951476746136;0.00133270803418135 0.00282479813276775 0.00133799988507366;0.00132951476746136 0.00133799988507366 0.00282448912315926]  Capacitance=[7.89543174552926e-09 -1.85986777702161e-09 -1.7901190036642e-09;-1.85986777702161e-09 7.82540023894543e-09 -1.8957321828871e-09;-1.7901190036642e-09 -1.8957321828871e-09 7.91264394645417e-09]  x1=[222.044860664132 9895.93129049812 9895.45603097759;314.159265358979 314.159265358979 314.159265358979;-3.07402242123169 -0.184553004701703 -1.7553903231323]  x2=[222.044785384515 9894.81350121358 9894.3402743402;314.159265358979 314.159265358979 314.159265358979;-3.07406302101548 -0.184588678342905 -1.75542561036529]  x3=[0.190189653397737 23.9020601443627 24.0934403694446;314.159265358979 314.159265358979 314.159265358979;-3.08343905277564 -0.165523944485925 -1.73654740167145]  x4=[0.197889836134495 26.4060462832311 26.5979715142426;314.159265358979 314.159265358979 314.159265358979;-3.06670973782009 -0.203121978729591 -1.7738046759858]  x5=5.51019361950282e-06  V1=ones(3,3)  V2=ones(3,3)  I1=ones(3,3)  I2=ones(3,3)  nHarmo=1  Measurements=None  Decoupling=off  VsMag0=0  VrMag0=0  VsAngle0=0  VrAngle0=0  IsMag0=0  IrMag0=0  IsAngle0=0  IrAngle0=0
      settings: SourceProductBaseCode=PS
  Line 55 : spsDistributedParametersLineLib/Distributed Parameters Line  Phases=3  Length=0.18999  Frequency=50  Resistance=[0.646656091154803 0.0486237908083191 0.0486712220507153;0.0486237908083191 0.646561225344642 0.0486237934466192;0.0486712220507153 0.0486237934466192 0.646656091154803]  Inductance=[0.00282448912315926 0.00133270803418135 0.00132951476746136;0.00133270803418135 0.00282479813276775 0.00133799988507366;0.00132951476746136 0.00133799988507366 0.00282448912315926]  Capacitance=[7.89543174552926e-09 -1.85986777702161e-09 -1.7901190036642e-09;-1.85986777702161e-09 7.82540023894543e-09 -1.8957321828871e-09;-1.7901190036642e-09 -1.8957321828871e-09 7.91264394645417e-09]  x1=[222.044785384515 9894.81350121358 9894.3402743402;314.159265358979 314.159265358979 314.159265358979;-3.07261793183714 -0.183440649901294 -1.7542764890819]  x2=[222.044700575796 9894.71596568863 9894.24290087527;314.159265358979 314.159265358979 314.159265358979;-3.07262122899411 -0.183443549243031 -1.754279352302]  x3=[0.192143151003701 24.5237168675502 24.7156692761455;314.159265358979 314.159265358979 314.159265358979;-3.07586021075732 -0.172913327735046 -1.74383642319737]  x4=[0.196105727679321 25.8302535343572 26.0224959761824;314.159265358979 314.159265358979 314.159265358979;-3.06972754008488 -0.193659759582689 -1.76441675893289]  x5=9.10331900668992e-07  V1=ones(3,3)  V2=ones(3,3)  I1=ones(3,3)  I2=ones(3,3)  nHarmo=1  Measurements=None  Decoupling=off  VsMag0=0  VrMag0=0  VsAngle0=0  VrAngle0=0  IsMag0=0  IrMag0=0  IsAngle0=0  IrAngle0=0
      settings: SourceProductBaseCode=PS
  Line 56 : spsDistributedParametersLineLib/Distributed Parameters Line  Phases=3  Length=0.34002  Frequency=50  Resistance=[0.646656091154803 0.0486237908083191 0.0486712220507153;0.0486237908083191 0.646561225344642 0.0486237934466192;0.0486712220507153 0.0486237934466192 0.646656091154803]  Inductance=[0.00282448912315926 0.00133270803418135 0.00132951476746136;0.00133270803418135 0.00282479813276775 0.00133799988507366;0.00132951476746136 0.00133799988507366 0.00282448912315926]  Capacitance=[7.89543174552926e-09 -1.85986777702161e-09 -1.7901190036642e-09;-1.85986777702161e-09 7.82540023894543e-09 -1.8957321828871e-09;-1.7901190036642e-09 -1.8957321828871e-09 7.91264394645417e-09]  x1=[222.044785384515 9894.81350121358 9894.3402743402;314.159265358979 314.159265358979 314.159265358979;-3.07284376982781 -0.183620063352295 -1.7544560733218]  x2=[222.044771263204 9894.65352200365 9894.18059853861;314.159265358979 314.159265358979 314.159265358979;-3.07284959403127 -0.183624903720532 -1.75446085967302]  x3=[0.19223986497943 24.5717688930877 24.7636624809618;314.159265358979 314.159265358979 314.159265358979;-3.07717461880694 -0.174197323093057 -1.74512278512913]  x4=[0.195982058436014 25.7729417534532 25.9651104308892;314.159265358979 314.159265358979 314.159265358979;-3.0691083541695 -0.193005551470305 -1.7637597938541]  x5=1.62919655174204e-06  V1=ones(3,3)  V2=ones(3,3)  I1=ones(3,3)  I2=ones(3,3)  nHarmo=1  Measurements=None  Decoupling=off  VsMag0=0  VrMag0=0  VsAngle0=0  VrAngle0=0  IsMag0=0  IrMag0=0  IsAngle0=0  IrAngle0=0
      settings: SourceProductBaseCode=PS
  Line 57 : spsDistributedParametersLineLib/Distributed Parameters Line  Phases=3  Length=0.12001  Frequency=50  Resistance=[0.646656091154803 0.0486237908083191 0.0486712220507153;0.0486237908083191 0.646561225344642 0.0486237934466192;0.0486712220507153 0.0486237934466192 0.646656091154803]  Inductance=[0.00282448912315926 0.00133270803418135 0.00132951476746136;0.00133270803418135 0.00282479813276775 0.00133799988507366;0.00132951476746136 0.00133799988507366 0.00282448912315926]  Capacitance=[7.89543174552926e-09 -1.85986777702161e-09 -1.7901190036642e-09;-1.85986777702161e-09 7.82540023894543e-09 -1.8957321828871e-09;-1.7901190036642e-09 -1.8957321828871e-09 7.91264394645417e-09]  x1=[222.044771263204 9894.65352200365 9894.18059853861;314.159265358979 314.159265358979 314.159265358979;-3.07251841615799 -0.183361804651315 -1.75419751015212]  x2=[222.044781926184 9894.63026896267 9894.15737105241;314.159265358979 314.159265358979 314.159265358979;-3.07251926417987 -0.183362952709189 -1.75419864851727]  x3=[0.193380911718643 24.9001994743594 25.0922845068636;314.159265358979 314.159265358979 314.159265358979;-3.07454771798343 -0.181041482207444 -1.75189794312194]  x4=[0.194880150284396 25.454600223219 25.6467889957714;314.159265358979 314.159265358979 314.159265358979;-3.07068552873078 -0.185774683603593 -1.75659058888102]  x5=5.75024640240464e-07  V1=ones(3,3)  V2=ones(3,3)  I1=ones(3,3)  I2=ones(3,3)  nHarmo=1  Measurements=None  Decoupling=off  VsMag0=0  VrMag0=0  VsAngle0=0  VrAngle0=0  IsMag0=0  IrMag0=0  IsAngle0=0  IrAngle0=0
      settings: SourceProductBaseCode=PS
  Line 58 : spsDistributedParametersLineLib/Distributed Parameters Line  Phases=3  Length=0.82  Frequency=50  Resistance=[0.646656091154803 0.0486237908083191 0.0486712220507153;0.0486237908083191 0.646561225344642 0.0486237934466192;0.0486712220507153 0.0486237934466192 0.646656091154803]  Inductance=[0.00282448912315926 0.00133270803418135 0.00132951476746136;0.00133270803418135 0.00282479813276775 0.00133799988507366;0.00132951476746136 0.00133799988507366 0.00282448912315926]  Capacitance=[7.89543174552926e-09 -1.85986777702161e-09 -1.7901190036642e-09;-1.85986777702161e-09 7.82540023894543e-09 -1.8957321828871e-09;-1.7901190036642e-09 -1.8957321828871e-09 7.91264394645417e-09]  x1=[222.044771263204 9894.65352200365 9894.18059853861;314.159265358979 314.159265358979 314.159265358979;-3.0735721009883 -0.184198888045075 -1.75503539038999]  x2=[222.044400319046 9894.41916936472 9893.94678919826;314.159265358979 314.159265358979 314.159265358979;-3.07357983962126 -0.184201762172957 -1.75503819239366]  x3=[0.192942772627685 24.834467457196 25.0262072801437;314.159265358979 314.159265358979 314.159265358979;-3.07533822678723 -0.176792605583138 -1.74769561160205]  x4=[0.195185261928763 25.4809864841476 25.6728947804872;314.159265358979 314.159265358979 314.159265358979;-3.0730613672562 -0.19238854667476 -1.76316251987548]  x5=3.92900762434114e-06  V1=ones(3,3)  V2=ones(3,3)  I1=ones(3,3)  I2=ones(3,3)  nHarmo=1  Measurements=None  Decoupling=off  VsMag0=0  VrMag0=0  VsAngle0=0  VrAngle0=0  IsMag0=0  IrMag0=0  IsAngle0=0  IrAngle0=0
      settings: SourceProductBaseCode=PS
  Line 59 : spsDistributedParametersLineLib/Distributed Parameters Line  Phases=3  Length=1.11  Frequency=50  Resistance=[0.646656091154803 0.0486237908083191 0.0486712220507153;0.0486237908083191 0.646561225344642 0.0486237934466192;0.0486712220507153 0.0486237934466192 0.646656091154803]  Inductance=[0.00282448912315926 0.00133270803418135 0.00132951476746136;0.00133270803418135 0.00282479813276775 0.00133799988507366;0.00132951476746136 0.00133799988507366 0.00282448912315926]  Capacitance=[7.89543174552926e-09 -1.85986777702161e-09 -1.7901190036642e-09;-1.85986777702161e-09 7.82540023894543e-09 -1.8957321828871e-09;-1.7901190036642e-09 -1.8957321828871e-09 7.91264394645417e-09]  x1=[222.020723483188 9898.49942617432 9898.02069734616;314.159265358979 314.159265358979 314.159265358979;-3.07385370569231 -0.184375684390437 -1.75521391762707]  x2=[222.044860664132 9895.93129049812 9895.45603097759;314.159265358979 314.159265358979 314.159265358979;-3.07396220980979 -0.184505170681573 -1.75534244357758]  x3=[0.188608945086964 21.8414811022816 22.0323200511982;314.159265358979 314.159265358979 314.159265358979;3.12764173010474 -0.153725046251096 -1.72494133068699]  x4=[0.200637184180737 28.4884163688831 28.6807921278617;314.159265358979 314.159265358979 314.159265358979;-2.99879712466954 -0.209160668984709 -1.77975625011192]  x5=5.31853471099837e-06  V1=ones(3,3)  V2=ones(3,3)  I1=ones(3,3)  I2=ones(3,3)  nHarmo=1  Measurements=None  Decoupling=off  VsMag0=0  VrMag0=0  VsAngle0=0  VrAngle0=0  IsMag0=0  IrMag0=0  IsAngle0=0  IrAngle0=0
      settings: SourceProductBaseCode=PS
  Line 6 : spsDistributedParametersLineLib/Distributed Parameters Line  Phases=3  Length=0.54002  Frequency=50  Resistance=[0.646656091154803 0.0486237908083191 0.0486712220507153;0.0486237908083191 0.646561225344642 0.0486237934466192;0.0486712220507153 0.0486237934466192 0.646656091154803]  Inductance=[0.00282448912315926 0.00133270803418135 0.00132951476746136;0.00133270803418135 0.00282479813276775 0.00133799988507366;0.00132951476746136 0.00133799988507366 0.00282448912315926]  Capacitance=[7.89543174552926e-09 -1.85986777702161e-09 -1.7901190036642e-09;-1.85986777702161e-09 7.82540023894543e-09 -1.8957321828871e-09;-1.7901190036642e-09 -1.8957321828871e-09 7.91264394645417e-09]  x1=[221.986588052248 9902.49457442833 9902.00819341533;314.159265358979 314.159265358979 314.159265358979;-3.07296562604528 -0.183459089421183 -1.75429808578545]  x2=[221.998599971118 9900.83919865606 9900.35614301331;314.159265358979 314.159265358979 314.159265358979;-3.07298440137673 -0.183545627301185 -1.75438405723769]  x3=[0.195364083508795 20.7453983385291 20.9374287359825;314.159265358979 314.159265358979 314.159265358979;-3.13750943136209 -0.142851465791625 -1.71435425880556]  x4=[0.193532620203 29.6504608291207 29.841900362528;314.159265358979 314.159265358979 314.159265358979;-3.00864584303494 -0.212489195277316 -1.78294246709757]  x5=2.58749109426427e-06  V1=ones(3,3)  V2=ones(3,3)  I1=ones(3,3)  I2=ones(3,3)  nHarmo=1  Measurements=None  Decoupling=off  VsMag0=0  VrMag0=0  VsAngle0=0  VrAngle0=0  IsMag0=0  IrMag0=0  IsAngle0=0  IrAngle0=0
      settings: SourceProductBaseCode=PS
  Line 60 : spsDistributedParametersLineLib/Distributed Parameters Line  Phases=3  Length=0.20999  Frequency=50  Resistance=[0.646656091154803 0.0486237908083191 0.0486712220507153;0.0486237908083191 0.646561225344642 0.0486237934466192;0.0486712220507153 0.0486237934466192 0.646656091154803]  Inductance=[0.00282448912315926 0.00133270803418135 0.00132951476746136;0.00133270803418135 0.00282479813276775 0.00133799988507366;0.00132951476746136 0.00133799988507366 0.00282448912315926]  Capacitance=[7.89543174552926e-09 -1.85986777702161e-09 -1.7901190036642e-09;-1.85986777702161e-09 7.82540023894543e-09 -1.8957321828871e-09;-1.7901190036642e-09 -1.8957321828871e-09 7.91264394645417e-09]  x1=[222.020723483188 9898.49942617432 9898.02069734616;314.159265358979 314.159265358979 314.159265358979;-3.07249893364681 -0.18329940697902 -1.75413661567577]  x2=[222.023998481021 9898.55008271221 9898.07102868956;314.159265358979 314.159265358979 314.159265358979;-3.07249913699654 -0.183305919258857 -1.75414312853859]  x3=[0.197439871352478 25.1898103130974 25.3819422108369;314.159265358979 314.159265358979 314.159265358979;-3.11157817665523 -0.203805292942352 -1.77449305008361]  x4=[0.191068312499897 25.1898959255057 25.3820073421348;314.159265358979 314.159265358979 314.159265358979;-3.03243740844023 -0.163051239281013 -1.73403812197785]  x5=1.00616135492121e-06  V1=ones(3,3)  V2=ones(3,3)  I1=ones(3,3)  I2=ones(3,3)  nHarmo=1  Measurements=None  Decoupling=off  VsMag0=0  VrMag0=0  VsAngle0=0  VrAngle0=0  IsMag0=0  IrMag0=0  IsAngle0=0  IrAngle0=0
      settings: SourceProductBaseCode=PS
  Line 61 : spsDistributedParametersLineLib/Distributed Parameters Line  Phases=3  Length=0.23001  Frequency=50  Resistance=[0.476003738225748 0.351747138225748 0.351747138225748;0.351747138225748 0.476003738225748 0.351747138225748;0.351747138225748 0.351747138225748 0.476003738225748]  Inductance=[0.000705954362986426 0.000459934243504405 0.000459934243504405;0.000459934243504405 0.000705954362986426 0.000459934243504405;0.000459934243504405 0.000459934243504405 0.000705954362986426]  Capacitance=[5.7561313269996e-07 -1.37543883484145e-07 -1.37543912800485e-07;-1.37543883484145e-07 5.75613027339387e-07 -1.37543875208088e-07;-1.37543912800485e-07 -1.37543875208088e-07 5.75613005057695e-07]  x1=[315.697915686212 9900.0334630943 9900.42206737047;314.159265358979 314.159265358979 314.159265358979;-2.7365699307748 -0.102331902965463 -1.67310962130347]  x2=[315.698318392546 9900.03799786774 9900.42660232121;314.159265358979 314.159265358979 314.159265358979;-2.73657287649785 -0.102332639372725 -1.67311035771061]  x3=[4.28030706318957 532.406006789624 532.426864117218;314.159265358979 314.159265358979 314.159265358979;-2.73816865662723 -0.103289408991778 -1.67406712725546]  x4=[4.28030706844169 532.406006884985 532.426864211953;314.159265358979 314.159265358979 314.159265358979;-2.73657287647707 -0.10233263937213 -1.67311035771063]  x5=5.08421409621804e-06  V1=ones(3,3)  V2=ones(3,3)  I1=ones(3,3)  I2=ones(3,3)  nHarmo=1  Measurements=None  Decoupling=off  VsMag0=0  VrMag0=0  VsAngle0=0  VrAngle0=0  IsMag0=0  IrMag0=0  IsAngle0=0  IrAngle0=0
      settings: SourceProductBaseCode=PS
  Line 62 : spsDistributedParametersLineLib/Distributed Parameters Line  Phases=3  Length=0.24001  Frequency=50  Resistance=[0.646656091154803 0.0486237908083191 0.0486712220507153;0.0486237908083191 0.646561225344642 0.0486237934466192;0.0486712220507153 0.0486237934466192 0.646656091154803]  Inductance=[0.00282448912315926 0.00133270803418135 0.00132951476746136;0.00133270803418135 0.00282479813276775 0.00133799988507366;0.00132951476746136 0.00133799988507366 0.00282448912315926]  Capacitance=[7.89543174552926e-09 -1.85986777702161e-09 -1.7901190036642e-09;-1.85986777702161e-09 7.82540023894543e-09 -1.8957321828871e-09;-1.7901190036642e-09 -1.8957321828871e-09 7.91264394645417e-09]  x1=[221.942233282415 9954.41206303633 9953.7487403836;314.159265358979 314.159265358979 314.159265358979;-3.0708911543861 -0.181114926377159 -1.75196781560589]  x2=[221.938102037244 9951.00721775662 9950.35750648769;314.159265358979 314.159265358979 314.159265358979;-3.07100604576828 -0.181236420096518 -1.75208848469724]  x3=[0.139074949329178 9.11193921642584 9.22831639474886;314.159265358979 314.159265358979 314.159265358979;3.11117074862956 0.584679472255165 -1.00607126787142]  x4=[0.250079512523316 44.5267102142633 44.6931440419819;314.159265358979 314.159265358979 314.159265358979;-3.01509041149181 -0.323667452421225 -1.89279049167461]  x5=1.1500013657538e-06  V1=ones(3,3)  V2=ones(3,3)  I1=ones(3,3)  I2=ones(3,3)  nHarmo=1  Measurements=None  Decoupling=off  VsMag0=0  VrMag0=0  VsAngle0=0  VrAngle0=0  IsMag0=0  IrMag0=0  IsAngle0=0  IrAngle0=0
      settings: SourceProductBaseCode=PS
  Line 63 : spsDistributedParametersLineLib/Distributed Parameters Line  Phases=3  Length=0.02  Frequency=50  Resistance=[0.646656091154803 0.0486237908083191 0.0486712220507153;0.0486237908083191 0.646561225344642 0.0486237934466192;0.0486712220507153 0.0486237934466192 0.646656091154803]  Inductance=[0.00282448912315926 0.00133270803418135 0.00132951476746136;0.00133270803418135 0.00282479813276775 0.00133799988507366;0.00132951476746136 0.00133799988507366 0.00282448912315926]  Capacitance=[7.89543174552926e-09 -1.85986777702161e-09 -1.7901190036642e-09;-1.85986777702161e-09 7.82540023894543e-09 -1.8957321828871e-09;-1.7901190036642e-09 -1.8957321828871e-09 7.91264394645417e-09]  x1=[221.942233282415 9954.41206303633 9953.7487403836;314.159265358979 314.159265358979 314.159265358979;-3.07055997651282 -0.180851827307942 -1.75170446608499]  x2=[221.942216515913 9954.40445924588 9953.74115361562;314.159265358979 314.159265358979 314.159265358979;-3.07056021315082 -0.180851903543892 -1.75170453986934]  x3=[0.192586861333001 24.9098508331839 25.1025945735226;314.159265358979 314.159265358979 314.159265358979;-3.0713231471446 -0.17003598649375 -1.74097374717187]  x4=[0.195513160154414 25.75761779536 25.9505735216614;314.159265358979 314.159265358979 314.159265358979;-3.06983834370928 -0.191335268958107 -1.76210814913169]  x5=9.5829454252223e-08  V1=ones(3,3)  V2=ones(3,3)  I1=ones(3,3)  I2=ones(3,3)  nHarmo=1  Measurements=None  Decoupling=off  VsMag0=0  VrMag0=0  VsAngle0=0  VrAngle0=0  IsMag0=0  IrMag0=0  IsAngle0=0  IrAngle0=0
      settings: SourceProductBaseCode=PS
  Line 64 : spsDistributedParametersLineLib/Distributed Parameters Line  Phases=3  Length=0.5  Frequency=50  Resistance=[0.646656091154803 0.0486237908083191 0.0486712220507153;0.0486237908083191 0.646561225344642 0.0486237934466192;0.0486712220507153 0.0486237934466192 0.646656091154803]  Inductance=[0.00282448912315926 0.00133270803418135 0.00132951476746136;0.00133270803418135 0.00282479813276775 0.00133799988507366;0.00132951476746136 0.00133799988507366 0.00282448912315926]  Capacitance=[7.89543174552926e-09 -1.85986777702161e-09 -1.7901190036642e-09;-1.85986777702161e-09 7.82540023894543e-09 -1.8957321828871e-09;-1.7901190036642e-09 -1.8957321828871e-09 7.91264394645417e-09]  x1=[221.95117302987 9961.69306170122 9961.00094605507;314.159265358979 314.159265358979 314.159265358979;-3.0710370792483 -0.181170755683022 -1.75202571420056]  x2=[221.942233282415 9954.41206303633 9953.7487403836;314.159265358979 314.159265358979 314.159265358979;-3.07128251357557 -0.181425835549495 -1.75227902074174]  x3=[0.137632727215565 9.00916396591077 9.11572120016098;314.159265358979 314.159265358979 314.159265358979;3.10793243105716 0.636615097703069 -0.955013885604208]  x4=[0.251527899934602 44.9806770642068 45.1467551962281;314.159265358979 314.159265358979 314.159265358979;-3.01485507715001 -0.328319569165953 -1.89744176437346]  x5=2.39573635630557e-06  V1=ones(3,3)  V2=ones(3,3)  I1=ones(3,3)  I2=ones(3,3)  nHarmo=1  Measurements=None  Decoupling=off  VsMag0=0  VrMag0=0  VsAngle0=0  VrAngle0=0  IsMag0=0  IrMag0=0  IsAngle0=0  IrAngle0=0
      settings: SourceProductBaseCode=PS
  Line 65 : spsDistributedParametersLineLib/Distributed Parameters Line  Phases=3  Length=0.23  Frequency=50  Resistance=[0.646656091154803 0.0486237908083191 0.0486712220507153;0.0486237908083191 0.646561225344642 0.0486237934466192;0.0486712220507153 0.0486237934466192 0.646656091154803]  Inductance=[0.00282448912315926 0.00133270803418135 0.00132951476746136;0.00133270803418135 0.00282479813276775 0.00133799988507366;0.00132951476746136 0.00133799988507366 0.00282448912315926]  Capacitance=[7.89543174552926e-09 -1.85986777702161e-09 -1.7901190036642e-09;-1.85986777702161e-09 7.82540023894543e-09 -1.8957321828871e-09;-1.7901190036642e-09 -1.8957321828871e-09 7.91264394645417e-09]  x1=[221.955329086998 9965.21034980222 9964.50473710622;314.159265358979 314.159265358979 314.159265358979;-3.07051184973591 -0.180724378274963 -1.75157990794547]  x2=[221.95117302987 9961.69306170122 9961.00094605507;314.159265358979 314.159265358979 314.159265358979;-3.07063065215051 -0.180847876047149 -1.75170252720613]  x3=[0.134960416198877 8.6333486640682 8.71922465900314;314.159265358979 314.159265358979 314.159265358979;3.09836693237342 0.743829611462154 -0.849909158456918]  x4=[0.254460403225754 46.0201521704117 46.1863204506788;314.159265358979 314.159265358979 314.159265358979;-3.01033632266098 -0.331282396316659 -1.90042417272379]  x5=1.10203872390056e-06  V1=ones(3,3)  V2=ones(3,3)  I1=ones(3,3)  I2=ones(3,3)  nHarmo=1  Measurements=None  Decoupling=off  VsMag0=0  VrMag0=0  VsAngle0=0  VrAngle0=0  IsMag0=0  IrMag0=0  IsAngle0=0  IrAngle0=0
      settings: SourceProductBaseCode=PS
  Line 66 : spsDistributedParametersLineLib/Distributed Parameters Line  Phases=3  Length=1.62  Frequency=50  Resistance=[0.80718830189013 0.0486237908083191 0.0486712220507153;0.0486237908083191 0.807093436079969 0.0486237934466192;0.0486712220507153 0.0486237934466192 0.80718830189013]  Inductance=[0.00279786707424938 0.00133270803418135 0.00132951476746136;0.00133270803418135 0.00279817608385787 0.00133799988507366;0.00132951476746136 0.00133799988507366 0.00279786707424938]  Capacitance=[7.73340098830622e-09 -1.79942827973291e-09 -1.73218055098733e-09;-1.79942827973291e-09 7.66505189233746e-09 -1.83375898618858e-09;-1.73218055098733e-09 -1.83375898618858e-09 7.749673531177e-09]  x1=[277.020513641768 9964.98211931216 9964.14487310868;314.159265358979 314.159265358979 314.159265358979;-2.8491918007332 -0.18668117457884 -1.75740121163218]  x2=[277.021268819298 9964.9823566033 9964.14515954927;314.159265358979 314.159265358979 314.159265358979;-2.84919417755254 -0.186684538393026 -1.75740459424522]  x3=[0.24111041472684 25.2245500090834 25.4143309324277;314.159265358979 314.159265358979 314.159265358979;-2.85169010670281 -0.188422840178062 -1.75914566776276]  x4=[0.241257107569525 25.2484275754165 25.438210955158;314.159265358979 314.159265358979 314.159265358979;-2.84911784049511 -0.18684314983049 -1.75756202745505]  x5=7.70442045759223e-06  V1=ones(3,3)  V2=ones(3,3)  I1=ones(3,3)  I2=ones(3,3)  nHarmo=1  Measurements=None  Decoupling=off  VsMag0=0  VrMag0=0  VsAngle0=0  VrAngle0=0  IsMag0=0  IrMag0=0  IsAngle0=0  IrAngle0=0
      settings: SourceProductBaseCode=PS
  Line 67 : spsDistributedParametersLineLib/Distributed Parameters Line  Phases=3  Length=0.54002  Frequency=50  Resistance=[0.646656091154803 0.0486237908083191 0.0486712220507153;0.0486237908083191 0.646561225344642 0.0486237934466192;0.0486712220507153 0.0486237934466192 0.646656091154803]  Inductance=[0.00282448912315926 0.00133270803418135 0.00132951476746136;0.00133270803418135 0.00282479813276775 0.00133799988507366;0.00132951476746136 0.00133799988507366 0.00282448912315926]  Capacitance=[7.89543174552926e-09 -1.85986777702161e-09 -1.7901190036642e-09;-1.85986777702161e-09 7.82540023894543e-09 -1.8957321828871e-09;-1.7901190036642e-09 -1.8957321828871e-09 7.91264394645417e-09]  x1=[221.964548942036 9973.45897651104 9972.72163219217;314.159265358979 314.159265358979 314.159265358979;-3.07069840352765 -0.180803388690571 -1.7516613161145]  x2=[221.955329086998 9965.21034980222 9964.50473710622;314.159265358979 314.159265358979 314.159265358979;-3.07097851836131 -0.181095115847976 -1.7519509984344]  x3=[0.134989357249375 8.59273393507922 8.67902644547996;314.159265358979 314.159265358979 314.159265358979;3.09350743188565 0.739187955907474 -0.854651168440119]  x4=[0.254489218231104 46.018950037318 46.1850143897895;314.159265358979 314.159265358979 314.159265358979;-3.008529904497 -0.330432716541661 -1.89956968061432]  x5=2.58749109426427e-06  V1=ones(3,3)  V2=ones(3,3)  I1=ones(3,3)  I2=ones(3,3)  nHarmo=1  Measurements=None  Decoupling=off  VsMag0=0  VrMag0=0  VsAngle0=0  VrAngle0=0  IsMag0=0  IrMag0=0  IsAngle0=0  IrAngle0=0
      settings: SourceProductBaseCode=PS
  Line 68 : spsDistributedParametersLineLib/Distributed Parameters Line  Phases=3  Length=0.13998  Frequency=50  Resistance=[0.646656091154803 0.0486237908083191 0.0486712220507153;0.0486237908083191 0.646561225344642 0.0486237934466192;0.0486712220507153 0.0486237934466192 0.646656091154803]  Inductance=[0.00282448912315926 0.00133270803418135 0.00132951476746136;0.00133270803418135 0.00282479813276775 0.00133799988507366;0.00132951476746136 0.00133799988507366 0.00282448912315926]  Capacitance=[7.89543174552926e-09 -1.85986777702161e-09 -1.7901190036642e-09;-1.85986777702161e-09 7.82540023894543e-09 -1.8957321828871e-09;-1.7901190036642e-09 -1.8957321828871e-09 7.91264394645417e-09]  x1=[221.964548942036 9973.45897651104 9972.72163219217;314.159265358979 314.159265358979 314.159265358979;-3.07009622909728 -0.180325000655257 -1.75118247268766]  x2=[221.965804678858 9973.27916209364 9972.54200461848;314.159265358979 314.159265358979 314.159265358979;-3.07010312278142 -0.180334019396714 -1.75119141632672]  x3=[0.190717820679729 23.5302091681334 23.7228188129848;314.159265358979 314.159265358979 314.159265358979;-3.10535171429692 -0.164287084142734 -1.73528987468082]  x4=[0.197631003707977 27.2296453911246 27.4229609585758;314.159265358979 314.159265358979 314.159265358979;-3.03628827243528 -0.194348281353892 -1.76509515548407]  x5=6.70710350311308e-07  V1=ones(3,3)  V2=ones(3,3)  I1=ones(3,3)  I2=ones(3,3)  nHarmo=1  Measurements=None  Decoupling=off  VsMag0=0  VrMag0=0  VsAngle0=0  VrAngle0=0  IsMag0=0  IrMag0=0  IsAngle0=0  IrAngle0=0
      settings: SourceProductBaseCode=PS
  Line 69 : spsDistributedParametersLineLib/Distributed Parameters Line  Phases=3  Length=0.14997  Frequency=50  Resistance=[0.476003738225748 0.351747138225748 0.351747138225748;0.351747138225748 0.476003738225748 0.351747138225748;0.351747138225748 0.351747138225748 0.476003738225748]  Inductance=[0.000705954362986426 0.000459934243504405 0.000459934243504405;0.000459934243504405 0.000705954362986426 0.000459934243504405;0.000459934243504405 0.000459934243504405 0.000705954362986426]  Capacitance=[5.7561313269996e-07 -1.37543883484145e-07 -1.37543912800485e-07;-1.37543883484145e-07 5.75613027339387e-07 -1.37543875208088e-07;-1.37543912800485e-07 -1.37543875208088e-07 5.75613005057695e-07]  x1=[316.399487295947 9974.78516586161 9974.89505839615;314.159265358979 314.159265358979 314.159265358979;-2.7317187600842 -0.0991129487525053 -1.66990606286872]  x2=[316.399658883045 9974.74432527759 9974.85421736186;314.159265358979 314.159265358979 314.159265358979;-2.73172001240214 -0.0991140731532646 -1.66990718726944]  x3=[4.29394655417122 534.792118595331 534.797968961607;314.159265358979 314.159265358979 314.159265358979;-2.73276083007844 -0.0984001475329847 -1.66919326149669]  x4=[4.2939465225203 538.48874315107 538.494634245861;314.159265358979 314.159265358979 314.159265358979;-2.73172000165193 -0.100444059541318 -1.67123717376028]  x5=3.31498451375949e-06  V1=ones(3,3)  V2=ones(3,3)  I1=ones(3,3)  I2=ones(3,3)  nHarmo=1  Measurements=None  Decoupling=off  VsMag0=0  VrMag0=0  VsAngle0=0  VrAngle0=0  IsMag0=0  IrMag0=0  IsAngle0=0  IrAngle0=0
      settings: SourceProductBaseCode=PS
  Line 7 : spsDistributedParametersLineLib/Distributed Parameters Line  Phases=3  Length=0.13997  Frequency=50  Resistance=[0.646656091154803 0.0486237908083191 0.0486712220507153;0.0486237908083191 0.646561225344642 0.0486237934466192;0.0486712220507153 0.0486237934466192 0.646656091154803]  Inductance=[0.00282448912315926 0.00133270803418135 0.00132951476746136;0.00133270803418135 0.00282479813276775 0.00133799988507366;0.00132951476746136 0.00133799988507366 0.00282448912315926]  Capacitance=[7.89543174552926e-09 -1.85986777702161e-09 -1.7901190036642e-09;-1.85986777702161e-09 7.82540023894543e-09 -1.8957321828871e-09;-1.7901190036642e-09 -1.8957321828871e-09 7.91264394645417e-09]  x1=[221.986588052248 9902.49457442833 9902.00819341533;314.159265358979 314.159265358979 314.159265358979;-3.07236343656205 -0.182980689427364 -1.75381923038871]  x2=[221.987428035661 9902.29893232256 9901.8129381134;314.159265358979 314.159265358979 314.159265358979;-3.07237009104937 -0.182984170363646 -1.75382264474063]  x3=[0.190247028279541 23.5680347042093 23.7596785721492;314.159265358979 314.159265358979 314.159265358979;-3.09963859333192 -0.145674367787324 -1.71682389719791]  x4=[0.198046157713751 26.8558710623831 27.0484687169975;314.159265358979 314.159265358979 314.159265358979;-3.04637570753283 -0.215878430888233 -1.78647521293591]  x5=6.70662435584182e-07  V1=ones(3,3)  V2=ones(3,3)  I1=ones(3,3)  I2=ones(3,3)  nHarmo=1  Measurements=None  Decoupling=off  VsMag0=0  VrMag0=0  VsAngle0=0  VrAngle0=0  IsMag0=0  IrMag0=0  IsAngle0=0  IrAngle0=0
      settings: SourceProductBaseCode=PS
  Line 70 : spsDistributedParametersLineLib/Distributed Parameters Line  Phases=3  Length=0.50001  Frequency=50  Resistance=[0.646656091154803 0.0486237908083191 0.0486712220507153;0.0486237908083191 0.646561225344642 0.0486237934466192;0.0486712220507153 0.0486237934466192 0.646656091154803]  Inductance=[0.00282448912315926 0.00133270803418135 0.00132951476746136;0.00133270803418135 0.00282479813276775 0.00133799988507366;0.00132951476746136 0.00133799988507366 0.00282448912315926]  Capacitance=[7.89543174552926e-09 -1.85986777702161e-09 -1.7901190036642e-09;-1.85986777702161e-09 7.82540023894543e-09 -1.8957321828871e-09;-1.7901190036642e-09 -1.8957321828871e-09 7.91264394645417e-09]  x1=[221.968468871425 9981.73540556523 9980.96799346069;314.159265358979 314.159265358979 314.159265358979;-3.07035391895599 -0.180453152697624 -1.75131318655554]  x2=[221.964548942036 9973.45897651104 9972.72163219217;314.159265358979 314.159265358979 314.159265358979;-3.0706381770529 -0.180755542711936 -1.75161342458989]  x3=[0.132564720778014 7.95862670433466 8.00095726496211;314.159265358979 314.159265358979 314.159265358979;3.03942156388298 0.951734565099693 -0.645704189240852]  x4=[0.258471363663691 47.9231752372611 48.0894885599687;314.159265358979 314.159265358979 314.159265358979;-2.98252616350816 -0.331858562239084 -1.90104680562752]  x5=2.3957842710327e-06  V1=ones(3,3)  V2=ones(3,3)  I1=ones(3,3)  I2=ones(3,3)  nHarmo=1  Measurements=None  Decoupling=off  VsMag0=0  VrMag0=0  VsAngle0=0  VrAngle0=0  IsMag0=0  IrMag0=0  IsAngle0=0  IrAngle0=0
      settings: SourceProductBaseCode=PS
  Line 71 : spsDistributedParametersLineLib/Distributed Parameters Line  Phases=3  Length=0.17001  Frequency=50  Resistance=[0.646656091154803 0.0486237908083191 0.0486712220507153;0.0486237908083191 0.646561225344642 0.0486237934466192;0.0486712220507153 0.0486237934466192 0.646656091154803]  Inductance=[0.00282448912315926 0.00133270803418135 0.00132951476746136;0.00133270803418135 0.00282479813276775 0.00133799988507366;0.00132951476746136 0.00133799988507366 0.00282448912315926]  Capacitance=[7.89543174552926e-09 -1.85986777702161e-09 -1.7901190036642e-09;-1.85986777702161e-09 7.82540023894543e-09 -1.8957321828871e-09;-1.7901190036642e-09 -1.8957321828871e-09 7.91264394645417e-09]  x1=[221.968468871425 9981.73540556523 9980.96799346069;314.159265358979 314.159265358979 314.159265358979;-3.06985717472536 -0.180058522031557 -1.75091818022902]  x2=[221.968311697706 9981.57114061828 9980.8040086814;314.159265358979 314.159265358979 314.159265358979;-3.06986269261904 -0.1800632173346 -1.7509228153502]  x3=[0.190338453252651 24.1797701607062 24.3725489641681;314.159265358979 314.159265358979 314.159265358979;-3.07560269688759 -0.159481819025321 -1.73051329222531]  x4=[0.197784759295464 26.6246649002749 26.817925814466;314.159265358979 314.159265358979 314.159265358979;-3.06458448236676 -0.198943933198055 -1.76966089149265]  x5=8.14598275871021e-07  V1=ones(3,3)  V2=ones(3,3)  I1=ones(3,3)  I2=ones(3,3)  nHarmo=1  Measurements=None  Decoupling=off  VsMag0=0  VrMag0=0  VsAngle0=0  VrAngle0=0  IsMag0=0  IrMag0=0  IsAngle0=0  IrAngle0=0
      settings: SourceProductBaseCode=PS
  Line 72 : spsDistributedParametersLineLib/Distributed Parameters Line  Phases=3  Length=0.27999  Frequency=50  Resistance=[0.646656091154803 0.0486237908083191 0.0486712220507153;0.0486237908083191 0.646561225344642 0.0486237934466192;0.0486712220507153 0.0486237934466192 0.646656091154803]  Inductance=[0.00282448912315926 0.00133270803418135 0.00132951476746136;0.00133270803418135 0.00282479813276775 0.00133799988507366;0.00132951476746136 0.00133799988507366 0.00282448912315926]  Capacitance=[7.89543174552926e-09 -1.85986777702161e-09 -1.7901190036642e-09;-1.85986777702161e-09 7.82540023894543e-09 -1.8957321828871e-09;-1.7901190036642e-09 -1.8957321828871e-09 7.91264394645417e-09]  x1=[221.97086404364 9986.63899000585 9985.85427005375;314.159265358979 314.159265358979 314.159265358979;-3.06985433759413 -0.180012965541733 -1.75087404861123]  x2=[221.968468871425 9981.73540556523 9980.96799346069;314.159265358979 314.159265358979 314.159265358979;-3.07002272602986 -0.180190041669902 -1.75104982506475]  x3=[0.129124874703009 8.00050961245991 8.00745391841322;314.159265358979 314.159265358979 314.159265358979;3.02607262750935 1.1156343630472 -0.482227851284917]  x4=[0.262324435335465 49.2352538455506 49.4014886172166;314.159265358979 314.159265358979 314.159265358979;-2.97852670282462 -0.337308112028278 -1.90651282546087]  x5=1.341564444804e-06  V1=ones(3,3)  V2=ones(3,3)  I1=ones(3,3)  I2=ones(3,3)  nHarmo=1  Measurements=None  Decoupling=off  VsMag0=0  VrMag0=0  VsAngle0=0  VrAngle0=0  IsMag0=0  IrMag0=0  IsAngle0=0  IrAngle0=0
      settings: SourceProductBaseCode=PS
  Line 73 : spsDistributedParametersLineLib/Distributed Parameters Line  Phases=3  Length=0.01  Frequency=50  Resistance=[0.646656091154803 0.0486237908083191 0.0486712220507153;0.0486237908083191 0.646561225344642 0.0486237934466192;0.0486712220507153 0.0486237934466192 0.646656091154803]  Inductance=[0.00282448912315926 0.00133270803418135 0.00132951476746136;0.00133270803418135 0.00282479813276775 0.00133799988507366;0.00132951476746136 0.00133799988507366 0.00282448912315926]  Capacitance=[7.89543174552926e-09 -1.85986777702161e-09 -1.7901190036642e-09;-1.85986777702161e-09 7.82540023894543e-09 -1.8957321828871e-09;-1.7901190036642e-09 -1.8957321828871e-09 7.91264394645417e-09]  x1=[221.970948975718 9986.81410936317 9986.02877112867;314.159265358979 314.159265358979 314.159265358979;-3.06944191011184 -0.179683774069546 -1.75054459615355]  x2=[221.97086404364 9986.63899000585 9985.85427005375;314.159265358979 314.159265358979 314.159265358979;-3.06944792554919 -0.179690097864365 -1.7505508735867]  x3=[0.129144944382544 8.00284589105329 8.00989402563968;314.159265358979 314.159265358979 314.159265358979;3.02647805313968 1.1155849430293 -0.482279197036921]  x4=[0.262368452473277 49.2582349207323 49.4246836298684;314.159265358979 314.159265358979 314.159265358979;-2.97768948296921 -0.336676502104634 -1.90588061970783]  x5=4.79147271261115e-08  V1=ones(3,3)  V2=ones(3,3)  I1=ones(3,3)  I2=ones(3,3)  nHarmo=1  Measurements=None  Decoupling=off  VsMag0=0  VrMag0=0  VsAngle0=0  VrAngle0=0  IsMag0=0  IrMag0=0  IsAngle0=0  IrAngle0=0
      settings: SourceProductBaseCode=PS
  Line 74 : spsDistributedParametersLineLib/Distributed Parameters Line  Phases=3  Length=0.04  Frequency=50  Resistance=[0.646656091154803 0.0486237908083191 0.0486712220507153;0.0486237908083191 0.646561225344642 0.0486237934466192;0.0486712220507153 0.0486237934466192 0.646656091154803]  Inductance=[0.00282448912315926 0.00133270803418135 0.00132951476746136;0.00133270803418135 0.00282479813276775 0.00133799988507366;0.00132951476746136 0.00133799988507366 0.00282448912315926]  Capacitance=[7.89543174552926e-09 -1.85986777702161e-09 -1.7901190036642e-09;-1.85986777702161e-09 7.82540023894543e-09 -1.8957321828871e-09;-1.7901190036642e-09 -1.8957321828871e-09 7.91264394645417e-09]  x1=[221.971288281389 9987.51457650419 9986.72676505534;314.159265358979 314.159265358979 314.159265358979;-3.06946300599794 -0.179694354803576 -1.75055539644594]  x2=[221.970948975718 9986.81410936316 9986.02877112867;314.159265358979 314.159265358979 314.159265358979;-3.06948706867826 -0.179719649584643 -1.75058050581959]  x3=[0.129144357077768 8.00251823402536 8.00959895166438;314.159265358979 314.159265358979 314.159265358979;3.02637859015791 1.11535012028728 -0.482515028715753]  x4=[0.262365404778276 49.2571918252087 49.4236261383258;314.159265358979 314.159265358979 314.159265358979;-2.97771881874773 -0.336702566903643 -1.90590670968489]  x5=1.91658908504446e-07  V1=ones(3,3)  V2=ones(3,3)  I1=ones(3,3)  I2=ones(3,3)  nHarmo=1  Measurements=None  Decoupling=off  VsMag0=0  VrMag0=0  VsAngle0=0  VrAngle0=0  IsMag0=0  IrMag0=0  IsAngle0=0  IrAngle0=0
      settings: SourceProductBaseCode=PS
  Line 8 : spsDistributedParametersLineLib/Distributed Parameters Line  Phases=3  Length=0.14997  Frequency=50  Resistance=[0.476003738225748 0.351747138225748 0.351747138225748;0.351747138225748 0.476003738225748 0.351747138225748;0.351747138225748 0.351747138225748 0.476003738225748]  Inductance=[0.000705954362986426 0.000459934243504405 0.000459934243504405;0.000459934243504405 0.000705954362986426 0.000459934243504405;0.000459934243504405 0.000459934243504405 0.000705954362986426]  Capacitance=[5.7561313269996e-07 -1.37543883484145e-07 -1.37543912800485e-07;-1.37543883484145e-07 5.75613027339387e-07 -1.37543875208088e-07;-1.37543912800485e-07 -1.37543875208088e-07 5.75613005057695e-07]  x1=[315.687816580921 9903.78369443125 9904.16368094112;314.159265358979 314.159265358979 314.159265358979;-2.73579240544846 -0.101760895878916 -1.67253979246357]  x2=[315.687987780165 9903.74087216881 9904.12085703534;314.159265358979 314.159265358979 314.159265358979;-2.73579365777193 -0.101760846758516 -1.67253974334312]  x3=[4.28428825779414 531.177713542553 531.198052506432;314.159265358979 314.159265358979 314.159265358979;-2.73683447646636 -0.100099262993717 -1.67087815935117]  x4=[4.28428825154423 534.464816900202 534.485281987158;314.159265358979 314.159265358979 314.159265358979;-2.73579364600108 -0.104034565584342 -1.67481346234567]  x5=3.31498451375949e-06  V1=ones(3,3)  V2=ones(3,3)  I1=ones(3,3)  I2=ones(3,3)  nHarmo=1  Measurements=None  Decoupling=off  VsMag0=0  VrMag0=0  VsAngle0=0  VrAngle0=0  IsMag0=0  IrMag0=0  IsAngle0=0  IrAngle0=0
      settings: SourceProductBaseCode=PS
  Line 9 : spsDistributedParametersLineLib/Distributed Parameters Line  Phases=3  Length=0.50001  Frequency=50  Resistance=[0.646656091154803 0.0486237908083191 0.0486712220507153;0.0486237908083191 0.646561225344642 0.0486237934466192;0.0486712220507153 0.0486237934466192 0.646656091154803]  Inductance=[0.00282448912315926 0.00133270803418135 0.00132951476746136;0.00133270803418135 0.00282479813276775 0.00133799988507366;0.00132951476746136 0.00133799988507366 0.00282448912315926]  Capacitance=[7.89543174552926e-09 -1.85986777702161e-09 -1.7901190036642e-09;-1.85986777702161e-09 7.82540023894543e-09 -1.8957321828871e-09;-1.7901190036642e-09 -1.8957321828871e-09 7.91264394645417e-09]  x1=[221.972317308412 9904.72208898904 9904.23123830907;314.159265358979 314.159265358979 314.159265358979;-3.0728639517429 -0.183318180125859 -1.75415788839096]  x2=[221.986588052248 9902.49457442834 9902.00819341533;314.159265358979 314.159265358979 314.159265358979;-3.07290539957053 -0.183411243442549 -1.75425019426083]  x3=[0.191887147541655 19.1666065432323 19.3573018110468;314.159265358979 314.159265358979 314.159265358979;3.11672015984651 -0.0941644930820911 -1.66621995785597]  x4=[0.197827794414034 31.3354108698259 31.526970022324;314.159265358979 314.159265358979 314.159265358979;-2.9828635546172 -0.238361021435807 -1.80866471684385]  x5=2.3957842710327e-06  V1=ones(3,3)  V2=ones(3,3)  I1=ones(3,3)  I2=ones(3,3)  nHarmo=1  Measurements=None  Decoupling=off  VsMag0=0  VrMag0=0  VsAngle0=0  VrAngle0=0  IsMag0=0  IrMag0=0  IsAngle0=0  IrAngle0=0
      settings: SourceProductBaseCode=PS
  Line im1 : spsDistributedParametersLineLib/Distributed Parameters Line  Phases=3  Length=1e-10  Frequency=50  Resistance=[0.646656091154803 0.0486237908083191 0.0486712220507153;0.0486237908083191 0.646561225344642 0.0486237934466192;0.0486712220507153 0.0486237934466192 0.646656091154803]  Inductance=[0.00282448912315926 0.00133270803418135 0.00132951476746136;0.00133270803418135 0.00282479813276775 0.00133799988507366;0.00132951476746136 0.00133799988507366 0.00282448912315926]  Capacitance=[7.89543174552926e-09 -1.85986777702161e-09 -1.7901190036642e-09;-1.85986777702161e-09 7.82540023894543e-09 -1.8957321828871e-09;-1.7901190036642e-09 -1.8957321828871e-09 7.91264394645417e-09]  x1=[222.020723483214 9898.49942617451 9898.02069734636;314.159265358979 314.159265358979 314.159265358979;-3.07218283873486 -0.18304829033195 -1.75388525998343]  x2=[222.020723483188 9898.49942617431 9898.02069734616;314.159265358979 314.159265358979 314.159265358979;-3.07218283873486 -0.183048290331965 -1.75388525998345]  x3=[0.191713160886326 22.0104714235727 22.1974398087936;314.159265358979 314.159265358979 314.159265358979;-2.41664777909391 -0.182571204952739 -1.74021175555027]  x4=[0.288377517715114 28.3494791544033 28.5628252315445;314.159265358979 314.159265358979 314.159265358979;2.77062667849612 -0.183351471256437 -1.76480023585486]  x5=4.79147271261115e-16  V1=ones(3,3)  V2=ones(3,3)  I1=ones(3,3)  I2=ones(3,3)  nHarmo=1  Measurements=None  Decoupling=off  VsMag0=0  VrMag0=0  VsAngle0=0  VrAngle0=0  IsMag0=0  IrMag0=0  IsAngle0=0  IrAngle0=0
      settings: SourceProductBaseCode=PS
  Line im2 : spsDistributedParametersLineLib/Distributed Parameters Line  Phases=3  Length=1e-10  Frequency=50  Resistance=[0.646656091154803 0.0486237908083191 0.0486712220507153;0.0486237908083191 0.646561225344642 0.0486237934466192;0.0486712220507153 0.0486237934466192 0.646656091154803]  Inductance=[0.00282448912315926 0.00133270803418135 0.00132951476746136;0.00133270803418135 0.00282479813276775 0.00133799988507366;0.00132951476746136 0.00133799988507366 0.00282448912315926]  Capacitance=[7.89543174552926e-09 -1.85986777702161e-09 -1.7901190036642e-09;-1.85986777702161e-09 7.82540023894543e-09 -1.8957321828871e-09;-1.7901190036642e-09 -1.8957321828871e-09 7.91264394645417e-09]  x1=[221.977087028903 9923.47138515495 9922.92903593915;314.159265358979 314.159265358979 314.159265358979;-3.07147469841167 -0.181975145418011 -1.75281748354344]  x2=[221.9770870289 9923.47138515393 9922.92903593815;314.159265358979 314.159265358979 314.159265358979;-3.07147469841171 -0.181975145418047 -1.75281748354348]  x3=[0.153170495134247 12.5239527528523 12.7840938960958;314.159265358979 314.159265358979 314.159265358979;-3.11462103654447 0.189140421680935 -1.41630925107007]  x4=[0.243663630769789 39.0855396208887 39.0383753975492;314.159265358979 314.159265358979 314.159265358979;-3.08288114335435 -0.298181354853508 -1.86135030742907]  x5=4.79147271261115e-16  V1=ones(3,3)  V2=ones(3,3)  I1=ones(3,3)  I2=ones(3,3)  nHarmo=1  Measurements=None  Decoupling=off  VsMag0=0  VrMag0=0  VsAngle0=0  VrAngle0=0  IsMag0=0  IrMag0=0  IsAngle0=0  IrAngle0=0
      settings: SourceProductBaseCode=PS
  Line im3 : spsDistributedParametersLineLib/Distributed Parameters Line  Phases=3  Length=1e-10  Frequency=50  Resistance=[0.646656091154803 0.0486237908083191 0.0486712220507153;0.0486237908083191 0.646561225344642 0.0486237934466192;0.0486712220507153 0.0486237934466192 0.646656091154803]  Inductance=[0.00282448912315926 0.00133270803418135 0.00132951476746136;0.00133270803418135 0.00282479813276775 0.00133799988507366;0.00132951476746136 0.00133799988507366 0.00282448912315926]  Capacitance=[7.89543174552926e-09 -1.85986777702161e-09 -1.7901190036642e-09;-1.85986777702161e-09 7.82540023894543e-09 -1.8957321828871e-09;-1.7901190036642e-09 -1.8957321828871e-09 7.91264394645417e-09]  x1=[221.938102037244 9951.00721775663 9950.35750648769;314.159265358979 314.159265358979 314.159265358979;-3.0706447621842 -0.180949404017356 -1.75180119539909]  x2=[221.938102037263 9951.00721775521 9950.35750648626;314.159265358979 314.159265358979 314.159265358979;-3.07064476218417 -0.180949404017406 -1.75180119539914]  x3=[0.275256536043535 9.21392599626689 9.399938475536;314.159265358979 314.159265358979 314.159265358979;2.92750269488388 0.586588514965317 -0.989855506802467]  x4=[0.150855564149645 44.4892789090256 44.7108606846684;314.159265358979 314.159265358979 314.159265358979;-2.53231538441649 -0.325378900968589 -1.89790251017971]  x5=4.79147271261115e-16  V1=ones(3,3)  V2=ones(3,3)  I1=ones(3,3)  I2=ones(3,3)  nHarmo=1  Measurements=None  Decoupling=off  VsMag0=0  VrMag0=0  VsAngle0=0  VrAngle0=0  IsMag0=0  IrMag0=0  IsAngle0=0  IrAngle0=0
      settings: SourceProductBaseCode=PS
  Line im4 : spsDistributedParametersLineLib/Distributed Parameters Line  Phases=3  Length=1e-10  Frequency=50  Resistance=[0.646656091154803 0.0486237908083191 0.0486712220507153;0.0486237908083191 0.646561225344642 0.0486237934466192;0.0486712220507153 0.0486237934466192 0.646656091154803]  Inductance=[0.00282448912315926 0.00133270803418135 0.00132951476746136;0.00133270803418135 0.00282479813276775 0.00133799988507366;0.00132951476746136 0.00133799988507366 0.00282448912315926]  Capacitance=[7.89543174552926e-09 -1.85986777702161e-09 -1.7901190036642e-09;-1.85986777702161e-09 7.82540023894543e-09 -1.8957321828871e-09;-1.7901190036642e-09 -1.8957321828871e-09 7.91264394645417e-09]  x1=[221.962982765956 9906.41761558302 9905.92344904595;314.159265358979 314.159265358979 314.159265358979;-3.07207601884629 -0.182651232887703 -1.75349095488537]  x2=[221.962982765951 9906.41761558249 9905.92344904545;314.159265358979 314.159265358979 314.159265358979;-3.07207601884641 -0.182651232887724 -1.75349095488539]  x3=[0.0695631806084122 18.1450603120893 18.709483059038;314.159265358979 314.159265358979 314.159265358979;2.64453021736418 -0.0594552840059383 -1.6438418507381]  x4=[0.340965552761306 32.4828479429469 32.2695788132999;314.159265358979 314.159265358979 314.159265358979;-2.99040251939659 -0.25151882088108 -1.81716305397081]  x5=4.79147271261115e-16  V1=ones(3,3)  V2=ones(3,3)  I1=ones(3,3)  I2=ones(3,3)  nHarmo=1  Measurements=None  Decoupling=off  VsMag0=0  VrMag0=0  VsAngle0=0  VrAngle0=0  IsMag0=0  IrMag0=0  IsAngle0=0  IrAngle0=0
      settings: SourceProductBaseCode=PS
  Load 1 : spsThreePhaseSeriesRLCLoadLib/Three-Phase Series RLC Load  LConnTagsString=A|B|C  Configuration=Delta  NominalVoltage=11000  Vabc=[1e3 1e3 1e3]  Vabcp=[1e3 1e3 1e3]  NominalFrequency=50  UnbalancedPower=off  ActivePower=15824.9152  InductivePower=2570.7506  CapacitivePower=0  Pabc=[10e3 9e3 11e3]  QLabc=[100 90 110]  QCabc=[100 90 110]  Pabcp=[10e3 9e3 11e3]  QLabcp=[100 90 110]  QCabcp=[100 90 110]  Measurements=None  LoadType=constant Z
  Load 10 : spsThreePhaseSeriesRLCLoadLib/Three-Phase Series RLC Load  LConnTagsString=A|B|C  Configuration=Delta  NominalVoltage=11000  Vabc=[1e3 1e3 1e3]  Vabcp=[1e3 1e3 1e3]  NominalFrequency=50  UnbalancedPower=off  ActivePower=4323.4359  InductivePower=828.0114  CapacitivePower=0  Pabc=[10e3 9e3 11e3]  QLabc=[100 90 110]  QCabc=[100 90 110]  Pabcp=[10e3 9e3 11e3]  QLabcp=[100 90 110]  QCabcp=[100 90 110]  Measurements=None  LoadType=constant Z
  Load 11 : spsThreePhaseSeriesRLCLoadLib/Three-Phase Series RLC Load  LConnTagsString=A|B|C  Configuration=Delta  NominalVoltage=11000  Vabc=[1e3 1e3 1e3]  Vabcp=[1e3 1e3 1e3]  NominalFrequency=50  UnbalancedPower=off  ActivePower=4738.1257  InductivePower=1053.1426  CapacitivePower=0  Pabc=[10e3 9e3 11e3]  QLabc=[100 90 110]  QCabc=[100 90 110]  Pabcp=[10e3 9e3 11e3]  QLabcp=[100 90 110]  QCabcp=[100 90 110]  Measurements=None  LoadType=constant Z
  Load 12 : spsThreePhaseSeriesRLCLoadLib/Three-Phase Series RLC Load  LConnTagsString=A|B|C  Configuration=Delta  NominalVoltage=11000  Vabc=[1e3 1e3 1e3]  Vabcp=[1e3 1e3 1e3]  NominalFrequency=50  UnbalancedPower=off  ActivePower=25139.8308  InductivePower=12493.4802  CapacitivePower=0  Pabc=[10e3 9e3 11e3]  QLabc=[100 90 110]  QCabc=[100 90 110]  Pabcp=[10e3 9e3 11e3]  QLabcp=[100 90 110]  QCabcp=[100 90 110]  Measurements=None  LoadType=constant Z
  Load 13 : spsThreePhaseSeriesRLCLoadLib/Three-Phase Series RLC Load  LConnTagsString=A|B|C  Configuration=Delta  NominalVoltage=11000  Vabc=[1e3 1e3 1e3]  Vabcp=[1e3 1e3 1e3]  NominalFrequency=50  UnbalancedPower=off  ActivePower=24079.2199  InductivePower=18013.1231  CapacitivePower=0  Pabc=[10e3 9e3 11e3]  QLabc=[100 90 110]  QCabc=[100 90 110]  Pabcp=[10e3 9e3 11e3]  QLabcp=[100 90 110]  QCabcp=[100 90 110]  Measurements=None  LoadType=constant Z
  Load 14 : spsThreePhaseSeriesRLCLoadLib/Three-Phase Series RLC Load  LConnTagsString=A|B|C  Configuration=Delta  NominalVoltage=11000  Vabc=[1e3 1e3 1e3]  Vabcp=[1e3 1e3 1e3]  NominalFrequency=50  UnbalancedPower=off  ActivePower=35772.577  InductivePower=9527.3426  CapacitivePower=0  Pabc=[10e3 9e3 11e3]  QLabc=[100 90 110]  QCabc=[100 90 110]  Pabcp=[10e3 9e3 11e3]  QLabcp=[100 90 110]  QCabcp=[100 90 110]  Measurements=None  LoadType=constant Z
  Load 15 : spsThreePhaseSeriesRLCLoadLib/Three-Phase Series RLC Load  LConnTagsString=A|B|C  Configuration=Delta  NominalVoltage=11000  Vabc=[1e3 1e3 1e3]  Vabcp=[1e3 1e3 1e3]  NominalFrequency=50  UnbalancedPower=off  ActivePower=211.4935  InductivePower=65.3278  CapacitivePower=0  Pabc=[10e3 9e3 11e3]  QLabc=[100 90 110]  QCabc=[100 90 110]  Pabcp=[10e3 9e3 11e3]  QLabcp=[100 90 110]  QCabcp=[100 90 110]  Measurements=None  LoadType=constant Z
  Load 2 : spsThreePhaseSeriesRLCLoadLib/Three-Phase Series RLC Load  LConnTagsString=A|B|C  Configuration=Delta  NominalVoltage=11000  Vabc=[1e3 1e3 1e3]  Vabcp=[1e3 1e3 1e3]  NominalFrequency=50  UnbalancedPower=off  ActivePower=31568.4315  InductivePower=8827.2212  CapacitivePower=0  Pabc=[10e3 9e3 11e3]  QLabc=[100 90 110]  QCabc=[100 90 110]  Pabcp=[10e3 9e3 11e3]  QLabcp=[100 90 110]  QCabcp=[100 90 110]  Measurements=None  LoadType=constant Z
  Load 3 : spsThreePhaseSeriesRLCLoadLib/Three-Phase Series RLC Load  LConnTagsString=A|B|C  Configuration=Delta  NominalVoltage=11000  Vabc=[1e3 1e3 1e3]  Vabcp=[1e3 1e3 1e3]  NominalFrequency=50  UnbalancedPower=off  ActivePower=17584.9589  InductivePower=11729.8078  CapacitivePower=0  Pabc=[10e3 9e3 11e3]  QLabc=[100 90 110]  QCabc=[100 90 110]  Pabcp=[10e3 9e3 11e3]  QLabcp=[100 90 110]  QCabcp=[100 90 110]  Measurements=None  LoadType=constant Z
  Load 4 : spsThreePhaseSeriesRLCLoadLib/Three-Phase Series RLC Load  LConnTagsString=A|B|C  Configuration=Delta  NominalVoltage=11000  Vabc=[1e3 1e3 1e3]  Vabcp=[1e3 1e3 1e3]  NominalFrequency=50  UnbalancedPower=off  ActivePower=196.6026  InductivePower=106.6891  CapacitivePower=0  Pabc=[10e3 9e3 11e3]  QLabc=[100 90 110]  QCabc=[100 90 110]  Pabcp=[10e3 9e3 11e3]  QLabcp=[100 90 110]  QCabcp=[100 90 110]  Measurements=None  LoadType=constant Z
  Load 5 : spsThreePhaseSeriesRLCLoadLib/Three-Phase Series RLC Load  LConnTagsString=A|B|C  Configuration=Delta  NominalVoltage=11000  Vabc=[1e3 1e3 1e3]  Vabcp=[1e3 1e3 1e3]  NominalFrequency=50  UnbalancedPower=off  ActivePower=4901.1451  InductivePower=3591.1627  CapacitivePower=0  Pabc=[10e3 9e3 11e3]  QLabc=[100 90 110]  QCabc=[100 90 110]  Pabcp=[10e3 9e3 11e3]  QLabcp=[100 90 110]  QCabcp=[100 90 110]  Measurements=None  LoadType=constant Z
  Load 6 : spsThreePhaseSeriesRLCLoadLib/Three-Phase Series RLC Load  LConnTagsString=A|B|C  Configuration=Delta  NominalVoltage=11000  Vabc=[1e3 1e3 1e3]  Vabcp=[1e3 1e3 1e3]  NominalFrequency=50  UnbalancedPower=off  ActivePower=22956.4549  InductivePower=6517.993  CapacitivePower=0  Pabc=[10e3 9e3 11e3]  QLabc=[100 90 110]  QCabc=[100 90 110]  Pabcp=[10e3 9e3 11e3]  QLabcp=[100 90 110]  QCabcp=[100 90 110]  Measurements=None  LoadType=constant Z
  Load 7 : spsThreePhaseSeriesRLCLoadLib/Three-Phase Series RLC Load  LConnTagsString=A|B|C  Configuration=Delta  NominalVoltage=11000  Vabc=[1e3 1e3 1e3]  Vabcp=[1e3 1e3 1e3]  NominalFrequency=50  UnbalancedPower=off  ActivePower=29652.8781  InductivePower=7066.1586  CapacitivePower=0  Pabc=[10e3 9e3 11e3]  QLabc=[100 90 110]  QCabc=[100 90 110]  Pabcp=[10e3 9e3 11e3]  QLabcp=[100 90 110]  QCabcp=[100 90 110]  Measurements=None  LoadType=constant Z
  Load 8 : spsThreePhaseSeriesRLCLoadLib/Three-Phase Series RLC Load  LConnTagsString=A|B|C  Configuration=Delta  NominalVoltage=11000  Vabc=[1e3 1e3 1e3]  Vabcp=[1e3 1e3 1e3]  NominalFrequency=50  UnbalancedPower=off  ActivePower=28013.8895  InductivePower=7060.1796  CapacitivePower=0  Pabc=[10e3 9e3 11e3]  QLabc=[100 90 110]  QCabc=[100 90 110]  Pabcp=[10e3 9e3 11e3]  QLabcp=[100 90 110]  QCabcp=[100 90 110]  Measurements=None  LoadType=constant Z
  Load 8041 : spsThreePhaseSeriesRLCLoadLib/Three-Phase Series RLC Load  LConnTagsString=A|B|C  Configuration=Delta  NominalVoltage=11000  Vabc=[1e3 1e3 1e3]  Vabcp=[1e3 1e3 1e3]  NominalFrequency=50  UnbalancedPower=off  ActivePower=20649.9338  InductivePower=4463.3699  CapacitivePower=0  Pabc=[10e3 9e3 11e3]  QLabc=[100 90 110]  QCabc=[100 90 110]  Pabcp=[10e3 9e3 11e3]  QLabcp=[100 90 110]  QCabcp=[100 90 110]  Measurements=None  LoadType=constant Z
  Load 8173 : spsThreePhaseSeriesRLCLoadLib/Three-Phase Series RLC Load  LConnTagsString=A|B|C  Configuration=Delta  NominalVoltage=11000  Vabc=[1e3 1e3 1e3]  Vabcp=[1e3 1e3 1e3]  NominalFrequency=50  UnbalancedPower=off  ActivePower=25425.5297  InductivePower=14333.9164  CapacitivePower=0  Pabc=[10e3 9e3 11e3]  QLabc=[100 90 110]  QCabc=[100 90 110]  Pabcp=[10e3 9e3 11e3]  QLabcp=[100 90 110]  QCabcp=[100 90 110]  Measurements=None  LoadType=constant Z
  Load 8287 : spsThreePhaseSeriesRLCLoadLib/Three-Phase Series RLC Load  LConnTagsString=A|B|C  Configuration=Delta  NominalVoltage=11000  Vabc=[1e3 1e3 1e3]  Vabcp=[1e3 1e3 1e3]  NominalFrequency=50  UnbalancedPower=off  ActivePower=23670.633  InductivePower=9378.53  CapacitivePower=0  Pabc=[10e3 9e3 11e3]  QLabc=[100 90 110]  QCabc=[100 90 110]  Pabcp=[10e3 9e3 11e3]  QLabcp=[100 90 110]  QCabcp=[100 90 110]  Measurements=None  LoadType=constant Z
  Load 8293 : spsThreePhaseSeriesRLCLoadLib/Three-Phase Series RLC Load  LConnTagsString=A|B|C  Configuration=Delta  NominalVoltage=11000  Vabc=[1e3 1e3 1e3]  Vabcp=[1e3 1e3 1e3]  NominalFrequency=50  UnbalancedPower=off  ActivePower=5471.4553  InductivePower=3135.0093  CapacitivePower=0  Pabc=[10e3 9e3 11e3]  QLabc=[100 90 110]  QCabc=[100 90 110]  Pabcp=[10e3 9e3 11e3]  QLabcp=[100 90 110]  QCabcp=[100 90 110]  Measurements=None  LoadType=constant Z
  Load 8424 : spsThreePhaseSeriesRLCLoadLib/Three-Phase Series RLC Load  LConnTagsString=A|B|C  Configuration=Delta  NominalVoltage=11000  Vabc=[1e3 1e3 1e3]  Vabcp=[1e3 1e3 1e3]  NominalFrequency=50  UnbalancedPower=off  ActivePower=10256.5743  InductivePower=6890.3861  CapacitivePower=0  Pabc=[10e3 9e3 11e3]  QLabc=[100 90 110]  QCabc=[100 90 110]  Pabcp=[10e3 9e3 11e3]  QLabcp=[100 90 110]  QCabcp=[100 90 110]  Measurements=None  LoadType=constant Z
  Load 8485 : spsThreePhaseSeriesRLCLoadLib/Three-Phase Series RLC Load  LConnTagsString=A|B|C  Configuration=Delta  NominalVoltage=11000  Vabc=[1e3 1e3 1e3]  Vabcp=[1e3 1e3 1e3]  NominalFrequency=50  UnbalancedPower=off  ActivePower=19228.399  InductivePower=11827.9017  CapacitivePower=0  Pabc=[10e3 9e3 11e3]  QLabc=[100 90 110]  QCabc=[100 90 110]  Pabcp=[10e3 9e3 11e3]  QLabcp=[100 90 110]  QCabcp=[100 90 110]  Measurements=None  LoadType=constant Z
  Load 8551 : spsThreePhaseSeriesRLCLoadLib/Three-Phase Series RLC Load  LConnTagsString=A|B|C  Configuration=Delta  NominalVoltage=11000  Vabc=[1e3 1e3 1e3]  Vabcp=[1e3 1e3 1e3]  NominalFrequency=50  UnbalancedPower=off  ActivePower=5501.3695  InductivePower=3706.7021  CapacitivePower=0  Pabc=[10e3 9e3 11e3]  QLabc=[100 90 110]  QCabc=[100 90 110]  Pabcp=[10e3 9e3 11e3]  QLabcp=[100 90 110]  QCabcp=[100 90 110]  Measurements=None  LoadType=constant Z
  Load 8605 : spsThreePhaseSeriesRLCLoadLib/Three-Phase Series RLC Load  LConnTagsString=A|B|C  Configuration=Delta  NominalVoltage=11000  Vabc=[1e3 1e3 1e3]  Vabcp=[1e3 1e3 1e3]  NominalFrequency=50  UnbalancedPower=off  ActivePower=207.2072  InductivePower=138.2115  CapacitivePower=0  Pabc=[10e3 9e3 11e3]  QLabc=[100 90 110]  QCabc=[100 90 110]  Pabcp=[10e3 9e3 11e3]  QLabcp=[100 90 110]  QCabcp=[100 90 110]  Measurements=None  LoadType=constant Z
  Load 8733 : spsThreePhaseSeriesRLCLoadLib/Three-Phase Series RLC Load  LConnTagsString=A|B|C  Configuration=Delta  NominalVoltage=11000  Vabc=[1e3 1e3 1e3]  Vabcp=[1e3 1e3 1e3]  NominalFrequency=50  UnbalancedPower=off  ActivePower=6315.8267  InductivePower=3746.7366  CapacitivePower=0  Pabc=[10e3 9e3 11e3]  QLabc=[100 90 110]  QCabc=[100 90 110]  Pabcp=[10e3 9e3 11e3]  QLabcp=[100 90 110]  QCabcp=[100 90 110]  Measurements=None  LoadType=constant Z
  Load 8737 : spsThreePhaseSeriesRLCLoadLib/Three-Phase Series RLC Load  LConnTagsString=A|B|C  Configuration=Delta  NominalVoltage=11000  Vabc=[1e3 1e3 1e3]  Vabcp=[1e3 1e3 1e3]  NominalFrequency=50  UnbalancedPower=off  ActivePower=13908.0577  InductivePower=4652.3346  CapacitivePower=0  Pabc=[10e3 9e3 11e3]  QLabc=[100 90 110]  QCabc=[100 90 110]  Pabcp=[10e3 9e3 11e3]  QLabcp=[100 90 110]  QCabcp=[100 90 110]  Measurements=None  LoadType=constant Z
  Load 9 : spsThreePhaseSeriesRLCLoadLib/Three-Phase Series RLC Load  LConnTagsString=A|B|C  Configuration=Delta  NominalVoltage=11000  Vabc=[1e3 1e3 1e3]  Vabcp=[1e3 1e3 1e3]  NominalFrequency=50  UnbalancedPower=off  ActivePower=162.0425  InductivePower=86.4319  CapacitivePower=0  Pabc=[10e3 9e3 11e3]  QLabc=[100 90 110]  QCabc=[100 90 110]  Pabcp=[10e3 9e3 11e3]  QLabcp=[100 90 110]  QCabcp=[100 90 110]  Measurements=None  LoadType=constant Z
  R{1..5} (5 alike) : spsThreePhaseVIMeasurementLib/Three-Phase V-I Measurement  VoltageMeasurement=phase-to-ground  SetLabelV=off  LabelV=Vabc  Vpu=off  VpuLL=off  CurrentMeasurement=yes  SetLabelI=off  LabelI=Iabc  Ipu=off  Pbase=100e6  Vbase=500e3  OutputType=Complex  PhasorSimulation=on  PSBequivalent=0
  Scope R{1..5} (5 alike) : Scope  NumInputPorts=2
  Source PC1_TT2 : spsThreePhaseSourceLib/Three-Phase Source  InternalConnection=Yn  VoltagePhases=off  Voltage=10000  PhaseAngle=0  Voltage_phases=[25e3 25e3 25e3]/sqrt(3)  PhaseAngles_phases=[0 -120 +120]  Frequency=50  NonIdealSource=on  SpecifyImpedance=off  Resistance=0.14  Inductance=0.0031831  ShortCircuitLevel=100e6  BaseVoltage=25e3  XRratio=7  BusType=swing  Pref=10e3  Qref=0  Prefabc=[10e3, 10e3, 10e3]  Qrefabc=[0, 0, 0]  Qmin=-inf  Qmax=inf
  Source Zn : spsSeriesRLCBranchLib/Series RLC Branch  LConnTagsString=__new0  RConnTagsString=__new0  BranchType=RL  Resistance=1e6  Inductance=3.1831e-06  SetiL0=off  InitialCurrent=0  Capacitance=0  Setx0=off  InitialVoltage=0  Measurements=None
  powergui : spspowerguiLib/powergui  Priority=1  SimulationMode=Phasor  SampleTime=50e-6  frequency=50  Iterations=50  frequencyindice=50  Pbase=100e6  ErrMax=1e-4  UnitsV=kV  UnitsW=MW  buscounter=0  FunctionMessages=off  echomessages=off  EnableUseOfTLC=off  CurrentSourceSwitches=off  DisableSnubberDevices=off  DisableRonSwitches=off  DisableVfSwitches=off  DisplayEquations=off  AutomaticDiscreteSolvers=off  SolverType=Tustin/Backward Euler (TBE)  Interpol=off  ExternalGateDelay=off  methode=off  Ts=10  x0status=blocks  SPID=off  SwTol=0  HookPort=off  NonlinearTolerance=1e-4  nMaxIteration=100  ContinueOnMaxIteration=off  RestoreLinks=warning  ResistiveCurrentMeasurement=off  Frange=[0:2:500]  Ylog=off  Xlog=on  ShowGrid=off  save=off  variable=ZData  structure=0  ZoomFFT=off  StartTime=0.0  cycles=1  DisplayStyle=1  fundamental=60  FreqAxis=off  MaxFrequency=1000  frequencyindicesteady=1  RmsSteady=1  display=off
  wires:
  R5/2 -> Scope R5/2
  R2/1 -> Scope R2/1
  R5/1 -> Scope R5/1
  R2/2 -> Scope R2/2
  R3/2 -> Scope R3/2
  R3/1 -> Scope R3/1
  R1/1 -> Scope R1/1
  R1/2 -> Scope R1/2
  R4/1 -> Scope R4/1
  R4/2 -> Scope R4/2
  connections:
  Source Zn/RConn1 -- Source PC1_TT2/LConn1
  Source Zn/LConn1 -- Ground/LConn1
  Line 46/RConn1 -- Line 47/LConn1
  Line 46/RConn2 -- Line 47/LConn2
  Line 46/RConn3 -- Line 47/LConn3
  Line 66/LConn1 -- Line 65/LConn1 -- Line 67/RConn1
  Line 66/LConn2 -- Line 65/LConn2 -- Line 67/RConn2
  Line 66/LConn3 -- Line 65/LConn3 -- Line 67/RConn3
  Line 58/LConn1 -- Line 57/LConn1 -- Line 56/RConn1
  Line 58/LConn2 -- Line 57/LConn2 -- Line 56/RConn2
  Line 58/LConn3 -- Line 57/LConn3 -- Line 56/RConn3
  Line 10/LConn1 -- Line 9/LConn1 -- Line 11/RConn1
  Line 10/LConn2 -- Line 9/LConn2 -- Line 11/RConn2
  Line 10/LConn3 -- Line 9/LConn3 -- Line 11/RConn3
  Line 54/LConn1 -- Line 53/LConn1 -- Line 59/RConn1
  Line 54/LConn2 -- Line 53/LConn2 -- Line 59/RConn2
  Line 54/LConn3 -- Line 53/LConn3 -- Line 59/RConn3
  Line 35/LConn1 -- Line 34/LConn1 -- Line 36/RConn1
  Line 35/LConn2 -- Line 34/LConn2 -- Line 36/RConn2
  Line 35/LConn3 -- Line 34/LConn3 -- Line 36/RConn3
  Line 68/LConn1 -- Line 67/LConn1 -- Line 70/RConn1
  Line 68/LConn2 -- Line 67/LConn2 -- Line 70/RConn2
  Line 68/LConn3 -- Line 67/LConn3 -- Line 70/RConn3
  Line 60/RConn1 -- Line 61/LConn1
  Line 60/RConn2 -- Line 61/LConn2
  Line 60/RConn3 -- Line 61/LConn3
  Line 68/RConn1 -- Line 69/LConn1
  Line 68/RConn2 -- Line 69/LConn2
  Line 68/RConn3 -- Line 69/LConn3
  Line 2/LConn1 -- Line 1/LConn1 -- Line 3/RConn1
  Line 2/LConn2 -- Line 1/LConn2 -- Line 3/RConn2
  Line 2/LConn3 -- Line 1/LConn3 -- Line 3/RConn3
  Line 46/LConn1 -- Load 8173/LConn1 -- Line 45/LConn1 -- Line 50/RConn1
  Line 46/LConn2 -- Load 8173/LConn2 -- Line 45/LConn2 -- Line 50/RConn2
  Line 46/LConn3 -- Load 8173/LConn3 -- Line 45/LConn3 -- Line 50/RConn3
  Line 13/LConn1 -- Line im4/RConn1
  Line 13/LConn2 -- Line im4/RConn2
  Line 13/LConn3 -- Line im4/RConn3
  Line 37/LConn1 -- Line 36/LConn1 -- Line 39/RConn1
  Line 37/LConn2 -- Line 36/LConn2 -- Line 39/RConn2
  Line 37/LConn3 -- Line 36/LConn3 -- Line 39/RConn3
  Load 3/LConn1 -- Line 3/LConn1 -- Line 4/RConn1
  Load 3/LConn2 -- Line 3/LConn2 -- Line 4/RConn2
  Load 3/LConn3 -- Line 3/LConn3 -- Line 4/RConn3
  Line 16/LConn1 -- Line 17/RConn1
  Line 16/LConn2 -- Line 17/RConn2
  Line 16/LConn3 -- Line 17/RConn3
  Line 12/LConn1 -- Line 13/RConn1
  Line 12/LConn2 -- Line 13/RConn2
  Line 12/LConn3 -- Line 13/RConn3
  Line 73/LConn1 -- Line 74/RConn1
  Line 73/LConn2 -- Line 74/RConn2
  Line 73/LConn3 -- Line 74/RConn3
  Line 7/LConn1 -- Line 6/LConn1 -- Line 9/RConn1
  Line 7/LConn2 -- Line 6/LConn2 -- Line 9/RConn2
  Line 7/LConn3 -- Line 6/LConn3 -- Line 9/RConn3
  Line 62/RConn1 -- R5/LConn1
  Line 62/RConn2 -- R5/LConn2
  Line 62/RConn3 -- R5/LConn3
  Line 5/LConn1 -- Line 4/LConn1 -- Line 6/RConn1
  Line 5/LConn2 -- Line 4/LConn2 -- Line 6/RConn2
  Line 5/LConn3 -- Line 4/LConn3 -- Line 6/RConn3
  Line 28/RConn1 -- Load 12/LConn1
  Line 28/RConn2 -- Load 12/LConn2
  Line 28/RConn3 -- Load 12/LConn3
  Line 28/LConn1 -- Line 39/LConn1 -- Line 29/RConn1
  Line 28/LConn2 -- Line 39/LConn2 -- Line 29/RConn2
  Line 28/LConn3 -- Line 39/LConn3 -- Line 29/RConn3
  Line 15/LConn1 -- Line 26/LConn1 -- Line 16/RConn1
  Line 15/LConn2 -- Line 26/LConn2 -- Line 16/RConn2
  Line 15/LConn3 -- Line 26/LConn3 -- Line 16/RConn3
  Source PC1_TT2/RConn1 -- R2/LConn1
  Source PC1_TT2/RConn2 -- R2/LConn2
  Source PC1_TT2/RConn3 -- R2/LConn3
  Load 14/LConn1 -- Line 33/LConn1 -- Line 34/RConn1
  Load 14/LConn2 -- Line 33/LConn2 -- Line 34/RConn2
  Load 14/LConn3 -- Line 33/LConn3 -- Line 34/RConn3
  Line 22/RConn1 -- Load 9/LConn1
  Line 22/RConn2 -- Load 9/LConn2
  Line 22/RConn3 -- Load 9/LConn3
  Load 5/LConn1 -- Line 2/RConn1
  Load 5/LConn2 -- Line 2/RConn2
  Load 5/LConn3 -- Line 2/RConn3
  Line 8/RConn1 -- Load 2/LConn1
  Line 8/RConn2 -- Load 2/LConn2
  Line 8/RConn3 -- Load 2/LConn3
  Line im2/LConn1 -- R1/RConn1
  Line im2/LConn2 -- R1/RConn2
  Line im2/LConn3 -- R1/RConn3
  Line 66/RConn1 -- Load 8605/LConn1
  Line 66/RConn2 -- Load 8605/LConn2
  Line 66/RConn3 -- Load 8605/LConn3
  Line 44/LConn1 -- Line 45/RConn1
  Line 44/LConn2 -- Line 45/RConn2
  Line 44/LConn3 -- Line 45/RConn3
  Line 19/LConn1 -- Line 14/LConn1 -- Line 20/RConn1
  Line 19/LConn2 -- Line 14/LConn2 -- Line 20/RConn2
  Line 19/LConn3 -- Line 14/LConn3 -- Line 20/RConn3
  Line 55/RConn1 -- Load 8424/LConn1
  Line 55/RConn2 -- Load 8424/LConn2
  Line 55/RConn3 -- Load 8424/LConn3
  Line 25/RConn1 -- Load 7/LConn1
  Line 25/RConn2 -- Load 7/LConn2
  Line 25/RConn3 -- Load 7/LConn3
  Line 11/LConn1 -- Line 12/RConn1
  Line 11/LConn2 -- Line 12/RConn2
  Line 11/LConn3 -- Line 12/RConn3
  Line 30/LConn1 -- Line 31/RConn1
  Line 30/LConn2 -- Line 31/RConn2
  Line 30/LConn3 -- Line 31/RConn3
  Line im3/LConn1 -- R5/RConn1
  Line im3/LConn2 -- R5/RConn2
  Line im3/LConn3 -- R5/RConn3
  Line 22/LConn1 -- Line 21/LConn1 -- Line 23/RConn1
  Line 22/LConn2 -- Line 21/LConn2 -- Line 23/RConn2
  Line 22/LConn3 -- Line 21/LConn3 -- Line 23/RConn3
  Line 5/RConn1 -- Load 4/LConn1
  Line 5/RConn2 -- Load 4/LConn2
  Line 5/RConn3 -- Load 4/LConn3
  Line im2/RConn1 -- Line 31/LConn1
  Line im2/RConn2 -- Line 31/LConn2
  Line im2/RConn3 -- Line 31/LConn3
  Line 51/RConn1 -- Line 50/LConn1
  Line 51/RConn2 -- Line 50/LConn2
  Line 51/RConn3 -- Line 50/LConn3
  Line 14/RConn1 -- R1/LConn1
  Line 14/RConn2 -- R1/LConn2
  Line 14/RConn3 -- R1/LConn3
  Line 24/LConn1 -- Line 23/LConn1 -- Line 26/RConn1
  Line 24/LConn2 -- Line 23/LConn2 -- Line 26/RConn2
  Line 24/LConn3 -- Line 23/LConn3 -- Line 26/RConn3
  Load 8485/LConn1 -- Line 64/LConn1 -- Line 65/RConn1
  Load 8485/LConn2 -- Line 64/LConn2 -- Line 65/RConn2
  Load 8485/LConn3 -- Line 64/LConn3 -- Line 65/RConn3
  Line 29/LConn1 -- Line 30/RConn1
  Line 29/LConn2 -- Line 30/RConn2
  Line 29/LConn3 -- Line 30/RConn3
  Load 10/LConn1 -- Line 19/RConn1
  Load 10/LConn2 -- Line 19/RConn2
  Load 10/LConn3 -- Line 19/RConn3
  Line 56/LConn1 -- Line 55/LConn1 -- Line 54/RConn1
  Line 56/LConn2 -- Line 55/LConn2 -- Line 54/RConn2
  Line 56/LConn3 -- Line 55/LConn3 -- Line 54/RConn3
  Line 63/LConn1 -- Line 62/LConn1 -- Line 64/RConn1
  Line 63/LConn2 -- Line 62/LConn2 -- Line 64/RConn2
  Line 63/LConn3 -- Line 62/LConn3 -- Line 64/RConn3
  Line 32/LConn1 -- Line 27/LConn1 -- Line 33/RConn1
  Line 32/LConn2 -- Line 27/LConn2 -- Line 33/RConn2
  Line 32/LConn3 -- Line 27/LConn3 -- Line 33/RConn3
  Line 7/RConn1 -- Line 8/LConn1
  Line 7/RConn2 -- Line 8/LConn2
  Line 7/RConn3 -- Line 8/LConn3
  Line 37/RConn1 -- Line 38/LConn1
  Line 37/RConn2 -- Line 38/LConn2
  Line 37/RConn3 -- Line 38/LConn3
  Load 8737/LConn1 -- Line 52/RConn1
  Load 8737/LConn2 -- Line 52/RConn2
  Load 8737/LConn3 -- Line 52/RConn3
  Line 57/RConn1 -- Load 8293/LConn1
  Line 57/RConn2 -- Load 8293/LConn2
  Line 57/RConn3 -- Load 8293/LConn3
  Line 58/RConn1 -- Load 8551/LConn1
  Line 58/RConn2 -- Load 8551/LConn2
  Line 58/RConn3 -- Load 8551/LConn3
  Line 35/RConn1 -- Load 15/LConn1
  Line 35/RConn2 -- Load 15/LConn2
  Line 35/RConn3 -- Load 15/LConn3
  Line 74/LConn1 -- R2/RConn1
  Line 74/LConn2 -- R2/RConn2
  Line 74/LConn3 -- R2/RConn3
  Load 8/LConn1 -- Line 20/LConn1 -- Line 21/RConn1
  Load 8/LConn2 -- Line 20/LConn2 -- Line 21/RConn2
  Load 8/LConn3 -- Line 20/LConn3 -- Line 21/RConn3
  Line im4/LConn1 -- R4/RConn1
  Line im4/LConn2 -- R4/RConn2
  Line im4/LConn3 -- R4/RConn3
  Line 71/RConn1 -- Load 8041/LConn1
  Line 71/RConn2 -- Load 8041/LConn2
